simulink model "PROCESSOR"  (R2022b)
settings: Solver=FixedStepDiscrete  StartTime=0.0  StopTime=700  FixedStep=0.1  RelTol=1e-3  EnableMultiTasking=on
(part 2 of 2)

== stateflow chart PROCESSOR/Chart ==
  state SET_UP
    CODE_START=uint32(1);
    MEMORY=uint64(zeros([1 65536],"uint64"));
    MEMORY=STORE_INSTRUCTIONS(MEMORY,CODE_START);
    STACK_MIN=1025;
    STACK_MAX=8192;
    MEM_MIN=8193;
    MEM_MAX=64512;
    INTERUPT_TABLE=64513;
    RIP=CODE_START;
    RSP=uint32(8192);
    RBP=uint32(0);
    RCF=uint32(0);
    R=uint32(zeros([1 31],"uint32"));
    xR8=uint64(0);
    xR10=uint64(0);
    xR11=uint64(0);
    xR12=uint64(0);
    xR13=uint64(0);
    xR14=uint64(0);
    xR15=uint64(0);
  state FETCH
    state S128
      xR8=128;
    state S129
      xR8=129;
      sum=GET_REG(xR13,0,32);
    (default) -> S128
    S128 -> 1001 [order 1] : [~(GET_REG(RCF,3,5)==0)]
    S128 -> 999 [order 2] : [(GET_REG(RCF,3,5)==0)]{xR11=LOAD(MEMORY, RIP), xR13=SET_REG(xR13,0,32,uint64(RIP)),
        |  xR14=SET_REG(xR14,0,32,8), xR12=SET_REG(xR12,0,1,0), xR12=SET_REG(xR12,1,2,0),
        |  xR10=SET_REG(xR10,0,16,129)}
    1004 -> S129
    S129 -> 1057 : {RIP=uint32(sum)}
  state HALT
    state S0
      xR8=0;
    (default) -> S0
  state MULT
    state S69
      xR8=69;
      s=GET_REG(xR13,0,32);
      y_m=GET_REG(xR15,0,32);
      y_mNeg=GET_REG(xR12,6,7);
    state S68
      xR8=68;
      x_m=GET_REG(xR11,0,32);
      y_m=GET_REG(xR15,0,32);
      x_mNeg=GET_REG(xR12,5,6);
      y_mNeg=GET_REG(xR12,6,7);
    state S67
      xR8=67;
      x_m=GET_REG(xR11,0,32);
      y_m=GET_REG(xR15,0,32);
      x_m31=GET_REG(xR11,31,32);
      y_m31=GET_REG(xR15,31,32);
    state X
      svd=GET_REG(xR10,16,32);
    state S70
      xR8=70;
      s=GET_REG(xR13,0,32);
    state S1
      xR8=1;
      x_m=GET_REG(xR11,0,32);
      y_m0=GET_REG(xR15,0,1);
      y_m1=GET_REG(xR15,1,2);
    state S2
      xR8=2;
      s=GET_REG(xR13,0,32);
      co=GET_REG(xR12,2,3);
      x_m=GET_REG(xR11,0,32);
      y_mi=GET_REG(xR15,xR8,xR8+1);
    state ADDER
    state S3
      xR8=3;
      s=GET_REG(xR13,0,32);
      co=GET_REG(xR12,2,3);
      x_m=GET_REG(xR11,0,32);
      y_mi=GET_REG(xR15,xR8,xR8+1);
    state S4
      xR8=4;
      s=GET_REG(xR13,0,32);
      co=GET_REG(xR12,2,3);
      x_m=GET_REG(xR11,0,32);
      y_mi=GET_REG(xR15,xR8,xR8+1);
    state S5
      xR8=5;
      s=GET_REG(xR13,0,32);
      co=GET_REG(xR12,2,3);
      x_m=GET_REG(xR11,0,32);
      y_mi=GET_REG(xR15,xR8,xR8+1);
    state S6
      xR8=6;
      s=GET_REG(xR13,0,32);
      co=GET_REG(xR12,2,3);
      x_m=GET_REG(xR11,0,32);
      y_mi=GET_REG(xR15,xR8,xR8+1);
    state S7
      xR8=7;
      s=GET_REG(xR13,0,32);
      co=GET_REG(xR12,2,3);
      x_m=GET_REG(xR11,0,32);
      y_mi=GET_REG(xR15,xR8,xR8+1);
    state S8
      xR8=8;
      s=GET_REG(xR13,0,32);
      co=GET_REG(xR12,2,3);
      x_m=GET_REG(xR11,0,32);
      y_mi=GET_REG(xR15,xR8,xR8+1);
    state S9
      xR8=9;
      s=GET_REG(xR13,0,32);
      co=GET_REG(xR12,2,3);
      x_m=GET_REG(xR11,0,32);
      y_mi=GET_REG(xR15,xR8,xR8+1);
    state S10
      xR8=10;
      s=GET_REG(xR13,0,32);
      co=GET_REG(xR12,2,3);
      x_m=GET_REG(xR11,0,32);
      y_mi=GET_REG(xR15,xR8,xR8+1);
    state S11
      xR8=11;
      s=GET_REG(xR13,0,32);
      co=GET_REG(xR12,2,3);
      x_m=GET_REG(xR11,0,32);
      y_mi=GET_REG(xR15,xR8,xR8+1);
    state S12
      xR8=12;
      s=GET_REG(xR13,0,32);
      co=GET_REG(xR12,2,3);
      x_m=GET_REG(xR11,0,32);
      y_mi=GET_REG(xR15,xR8,xR8+1);
    state S13
      xR8=13;
      s=GET_REG(xR13,0,32);
      co=GET_REG(xR12,2,3);
      x_m=GET_REG(xR11,0,32);
      y_mi=GET_REG(xR15,xR8,xR8+1);
    state S14
      xR8=14;
      s=GET_REG(xR13,0,32);
      co=GET_REG(xR12,2,3);
      x_m=GET_REG(xR11,0,32);
      y_mi=GET_REG(xR15,xR8,xR8+1);
    state S15
      xR8=15;
      s=GET_REG(xR13,0,32);
      co=GET_REG(xR12,2,3);
      x_m=GET_REG(xR11,0,32);
      y_mi=GET_REG(xR15,xR8,xR8+1);
    state S16
      xR8=16;
      s=GET_REG(xR13,0,32);
      co=GET_REG(xR12,2,3);
      x_m=GET_REG(xR11,0,32);
      y_mi=GET_REG(xR15,xR8,xR8+1);
    state S17
      xR8=17;
      s=GET_REG(xR13,0,32);
      co=GET_REG(xR12,2,3);
      x_m=GET_REG(xR11,0,32);
      y_mi=GET_REG(xR15,xR8,xR8+1);
    state S18
      xR8=18;
      s=GET_REG(xR13,0,32);
      co=GET_REG(xR12,2,3);
      x_m=GET_REG(xR11,0,32);
      y_mi=GET_REG(xR15,xR8,xR8+1);
    state S19
      xR8=19;
      s=GET_REG(xR13,0,32);
      co=GET_REG(xR12,2,3);
      x_m=GET_REG(xR11,0,32);
      y_mi=GET_REG(xR15,xR8,xR8+1);
    state S20
      xR8=20;
      s=GET_REG(xR13,0,32);
      co=GET_REG(xR12,2,3);
      x_m=GET_REG(xR11,0,32);
      y_mi=GET_REG(xR15,xR8,xR8+1);
    state S21
      xR8=21;
      s=GET_REG(xR13,0,32);
      co=GET_REG(xR12,2,3);
      x_m=GET_REG(xR11,0,32);
      y_mi=GET_REG(xR15,xR8,xR8+1);
    state S22
      xR8=22;
      s=GET_REG(xR13,0,32);
      co=GET_REG(xR12,2,3);
      x_m=GET_REG(xR11,0,32);
      y_mi=GET_REG(xR15,xR8,xR8+1);
    state S23
      xR8=23;
      s=GET_REG(xR13,0,32);
      co=GET_REG(xR12,2,3);
      x_m=GET_REG(xR11,0,32);
      y_mi=GET_REG(xR15,xR8,xR8+1);
    state S24
      xR8=24;
      s=GET_REG(xR13,0,32);
      co=GET_REG(xR12,2,3);
      x_m=GET_REG(xR11,0,32);
      y_mi=GET_REG(xR15,xR8,xR8+1);
    state S25
      xR8=25;
      s=GET_REG(xR13,0,32);
      co=GET_REG(xR12,2,3);
      x_m=GET_REG(xR11,0,32);
      y_mi=GET_REG(xR15,xR8,xR8+1);
    state S26
      xR8=26;
      s=GET_REG(xR13,0,32);
      co=GET_REG(xR12,2,3);
      x_m=GET_REG(xR11,0,32);
      y_mi=GET_REG(xR15,xR8,xR8+1);
    state S27
      xR8=27;
      s=GET_REG(xR13,0,32);
      co=GET_REG(xR12,2,3);
      x_m=GET_REG(xR11,0,32);
      y_mi=GET_REG(xR15,xR8,xR8+1);
    state S28
      xR8=28;
      s=GET_REG(xR13,0,32);
      co=GET_REG(xR12,2,3);
      x_m=GET_REG(xR11,0,32);
      y_mi=GET_REG(xR15,xR8,xR8+1);
    state S29
      xR8=29;
      s=GET_REG(xR13,0,32);
      co=GET_REG(xR12,2,3);
      x_m=GET_REG(xR11,0,32);
      y_mi=GET_REG(xR15,xR8,xR8+1);
    state S30
      xR8=30;
      s=GET_REG(xR13,0,32);
      co=GET_REG(xR12,2,3);
      x_m=GET_REG(xR11,0,32);
      y_mi=GET_REG(xR15,xR8,xR8+1);
    state S31
      xR8=31;
      s=GET_REG(xR13,0,32);
      co=GET_REG(xR12,2,3);
      x_m=GET_REG(xR11,0,32);
      y_mi=GET_REG(xR15,xR8,xR8+1);
    state S71
      xR8=71;
      s=GET_REG(xR13,0,32);
      s31=GET_REG(xR13,31,32);
      co=GET_REG(xR12,2,3);
      x_mNeg=GET_REG(xR12,5,6);
      y_mNeg=GET_REG(xR12,6,7);
    state S73
      xR8=73;
      s=GET_REG(xR13,0,32);
      s31=GET_REG(xR13,31,32);
    state S72
      xR8=72;
    (junction 787) -> (junction 788)
    S67 -> (junction 787) [order 1] : [(y_m==1) & x_m & ~(x_m==1)]{
        | xR13=SET_REG(xR13,0,32,x_m),
        | xR12=SET_REG(xR12,7,8,x_m31),
        | xR12=SET_REG(xR12,8,9,0),
        | xR12=SET_REG(xR12,9,10,0)}
    (junction 788) -> (junction 790)
    (junction 802) -> (junction 804)
    (junction 795) -> (junction 802)
    (junction 800) -> (junction 795)
    S69 -> (junction 802) [order 1] : [y_mNeg]{
        | xR11=SET_REG(xR11,0,32,s),
        | xR13=SET_REG(xR13,0,32,0),
        | xR14=SET_REG(xR14,0,32,y_m),
        | xR12=SET_REG(xR12,1,2,0),
        | xR12=SET_REG(xR12,0,1,1),
        | xR10=SET_REG(xR10,0,16,70)}
    (junction 804) -> MULT.ADDER
    S68 -> (junction 795) [order 2] : [x_mNeg]{
        | xR13=SET_REG(xR13,0,32,0),
        | xR14=SET_REG(xR14,0,32,x_m),
        | xR12=SET_REG(xR12,1,2,0),
        | xR12=SET_REG(xR12,0,1,1),
        | xR10=SET_REG(xR10,0,16,69)}
    S68 -> (junction 800) [order 1] : [~x_mNeg & y_mNeg]{
        | xR13=SET_REG(xR13,0,32,0),
        | xR14=SET_REG(xR14,0,32,y_m),
        | xR12=SET_REG(xR12,1,2,0),
        | xR12=SET_REG(xR12,0,1,1),
        | xR10=SET_REG(xR10,0,16,70)}
    (junction 786) -> (junction 790)
    S67 -> (junction 786) [order 2] : [(x_m==1) & y_m & ~(y_m==1)]{
        | xR13=SET_REG(xR13,0,32,y_m),
        | xR12=SET_REG(xR12,7,8,y_m31),
        | xR12=SET_REG(xR12,8,9,0),
        | xR12=SET_REG(xR12,9,10,0)}
    (junction 790) -> MULT.X
    MULT.X -> 1377 [order 1] : [svd==195]
    MULT.X -> 1379 [order 2] : [svd==197]
    (default) -> S67
    447 -> S69
    S67 -> MULT.X [order 3] : [~x_m | ~y_m]{
        | xR13=SET_REG(xR13,0,32,0),
        | xR12=SET_REG(xR12,7,8,0),
        | xR12=SET_REG(xR12,8,9,0),
        | xR12=SET_REG(xR12,9,10,1)}
    S67 -> S68 [order 4] : [x_m & y_m & ~(x_m==1) & ~(y_m==1)]{
        | xR12=SET_REG(xR12,5,6,x_m31),
        | xR12=SET_REG(xR12,6,7,y_m31)}
    S73 -> MULT.X : {xR12=SET_REG(xR12,7,8,s31),
        | xR12=SET_REG(xR12,8,9,0)
        | xR12=SET_REG(xR12,9,10,~s)}
    S69 -> (junction 796) [order 2] : [~y_mNeg]{
        | xR11=SET_REG(xR11,0,32,s)}
    (junction 796) -> (junction 797)
    S68 -> S1 [order 3] : [~x_mNeg & ~y_mNeg]
    (junction 780) -> (junction 781)
    S1 -> (junction 780) [order 1] : [~y_m0 & ~y_m1]{
        | xR13=SET_REG(xR13,0,32,0)}
    (junction 781) -> (junction 779)
    (junction 778) -> (junction 779)
    S1 -> (junction 778) [order 2] : [~y_m0 & y_m1]{
        | xR13=SET_REG(xR13,0,32,bitsll(uint32(x_m),1))}
    (junction 779) -> S2
    453 -> S70
    463 -> S2
    (junction 797) -> S1
    S1 -> S2 [order 4] : [y_m0 & ~y_m1]{
        | xR13=SET_REG(xR13,0,32,x_m)}
    S70 -> S1 : {xR15=SET_REG(xR15,0,32,s)}
    S2 -> (junction 770) [order 3] : [(s | co)  & y_mi]{
        | xR14=SET_REG(xR14,0,32,bitsll(uint32(x_m),xR8)),
        | xR12=SET_REG(xR12,0,1,0),
        | xR12=SET_REG(xR12,1,2,co),
        | xR10=SET_REG(xR10,0,16,3)}
    (junction 770) -> (junction 771)
    S2 -> S3 [order 2] : [~s & ~co  & y_mi]{
        | xR13=SET_REG(xR13,0,32,bitsll(uint32(x_m),xR8))}
    S2 -> S3 [order 4] : [~s & ~co  & ~y_mi]{
        | xR13=SET_REG(xR13,0,32,0)}
    S1 -> (junction 768) [order 3] : [y_m0 & y_m1]{
        | xR13=SET_REG(xR13,0,32,x_m),
        | xR14=SET_REG(xR14,0,32,bitsll(uint32(x_m),1)),
        | xR12=SET_REG(xR12,0,1,0),
        | xR12=SET_REG(xR12,1,2,0),
        | xR10=SET_REG(xR10,0,16,2)}
    S2 -> (junction 772) [order 1] : [(s | co)  & ~y_mi]{
        | xR14=SET_REG(xR14,0,32,0),
        | xR12=SET_REG(xR12,0,1,0),
        | xR12=SET_REG(xR12,1,2,co),
        | xR10=SET_REG(xR10,0,16,3)}
    (junction 768) -> (junction 769)
    (junction 771) -> (junction 768)
    (junction 772) -> (junction 771)
    (junction 769) -> MULT.ADDER
    S3 -> MULT.ADDER [order 4] : [(s | co)  & y_mi]{
        | xR14=SET_REG(xR14,0,32,bitsll(uint32(x_m),xR8)),
        | xR12=SET_REG(xR12,0,1,0),
        | xR12=SET_REG(xR12,1,2,co),
        | xR10=SET_REG(xR10,0,16,4)}
    473 -> S3
    S3 -> MULT.ADDER [order 3] : [(s | co)  & ~y_mi]{
        | xR14=SET_REG(xR14,0,32,0),
        | xR12=SET_REG(xR12,0,1,0),
        | xR12=SET_REG(xR12,1,2,co),
        | xR10=SET_REG(xR10,0,16,4)}
    S3 -> S4 [order 2] : [~s & ~co  & y_mi]{
        | xR13=SET_REG(xR13,0,32,bitsll(uint32(x_m),xR8))}
    S3 -> S4 [order 1] : [~s & ~co  & ~y_mi]{
        | xR13=SET_REG(xR13,0,32,0)}
    MULT.ADDER -> 765
    S4 -> MULT.ADDER [order 4] : [(s | co)  & y_mi]{
        | xR14=SET_REG(xR14,0,32,bitsll(uint32(x_m),xR8)),
        | xR12=SET_REG(xR12,0,1,0),
        | xR12=SET_REG(xR12,1,2,co),
        | xR10=SET_REG(xR10,0,16,5)}
    483 -> S4
    S4 -> MULT.ADDER [order 3] : [(s | co)  & ~y_mi]{
        | xR14=SET_REG(xR14,0,32,0),
        | xR12=SET_REG(xR12,0,1,0),
        | xR12=SET_REG(xR12,1,2,co),
        | xR10=SET_REG(xR10,0,16,5)}
    S4 -> S5 [order 1] : [~s & ~co  & y_mi]{
        | xR13=SET_REG(xR13,0,32,bitsll(uint32(x_m),xR8))}
    S4 -> S5 [order 2] : [~s & ~co  & ~y_mi]{
        | xR13=SET_REG(xR13,0,32,0)}
    S5 -> MULT.ADDER [order 4] : [(s | co)  & y_mi]{
        | xR14=SET_REG(xR14,0,32,bitsll(uint32(x_m),xR8)),
        | xR12=SET_REG(xR12,0,1,0),
        | xR12=SET_REG(xR12,1,2,co),
        | xR10=SET_REG(xR10,0,16,6)}
    498 -> S5
    S5 -> MULT.ADDER [order 3] : [(s | co)  & ~y_mi]{
        | xR14=SET_REG(xR14,0,32,0),
        | xR12=SET_REG(xR12,0,1,0),
        | xR12=SET_REG(xR12,1,2,co),
        | xR10=SET_REG(xR10,0,16,6)}
    S5 -> S6 [order 2] : [~s & ~co  & y_mi]{
        | xR13=SET_REG(xR13,0,32,bitsll(uint32(x_m),xR8))}
    S5 -> S6 [order 1] : [~s & ~co  & ~y_mi]{
        | xR13=SET_REG(xR13,0,32,0)}
    S6 -> MULT.ADDER [order 4] : [(s | co)  & y_mi]{
        | xR14=SET_REG(xR14,0,32,bitsll(uint32(x_m),xR8)),
        | xR12=SET_REG(xR12,0,1,0),
        | xR12=SET_REG(xR12,1,2,co),
        | xR10=SET_REG(xR10,0,16,7)}
    496 -> S6
    S6 -> MULT.ADDER [order 3] : [(s | co)  & ~y_mi]{
        | xR14=SET_REG(xR14,0,32,0),
        | xR12=SET_REG(xR12,0,1,0),
        | xR12=SET_REG(xR12,1,2,co),
        | xR10=SET_REG(xR10,0,16,7)}
    S6 -> S7 [order 2] : [~s & ~co  & y_mi]{
        | xR13=SET_REG(xR13,0,32,bitsll(uint32(x_m),xR8))}
    S6 -> S7 [order 1] : [~s & ~co  & ~y_mi]{
        | xR13=SET_REG(xR13,0,32,0)}
    S7 -> MULT.ADDER [order 4] : [(s | co)  & y_mi]{
        | xR14=SET_REG(xR14,0,32,bitsll(uint32(x_m),xR8)),
        | xR12=SET_REG(xR12,0,1,0),
        | xR12=SET_REG(xR12,1,2,co),
        | xR10=SET_REG(xR10,0,16,8)}
    524 -> S7
    S7 -> MULT.ADDER [order 3] : [(s | co)  & ~y_mi]{
        | xR14=SET_REG(xR14,0,32,0),
        | xR12=SET_REG(xR12,0,1,0),
        | xR12=SET_REG(xR12,1,2,co),
        | xR10=SET_REG(xR10,0,16,8)}
    S7 -> S8 [order 2] : [~s & ~co  & y_mi]{
        | xR13=SET_REG(xR13,0,32,bitsll(uint32(x_m),xR8))}
    S7 -> S8 [order 1] : [~s & ~co  & ~y_mi]{
        | xR13=SET_REG(xR13,0,32,0)}
    S8 -> MULT.ADDER [order 4] : [(s | co)  & y_mi]{
        | xR14=SET_REG(xR14,0,32,bitsll(uint32(x_m),xR8)),
        | xR12=SET_REG(xR12,0,1,0),
        | xR12=SET_REG(xR12,1,2,co),
        | xR10=SET_REG(xR10,0,16,9)}
    S8 -> MULT.ADDER [order 3] : [(s | co)  & ~y_mi]{
        | xR14=SET_REG(xR14,0,32,0),
        | xR12=SET_REG(xR12,0,1,0),
        | xR12=SET_REG(xR12,1,2,co),
        | xR10=SET_REG(xR10,0,16,9)}
    522 -> S8
    S8 -> S9 [order 1] : [~s & ~co  & y_mi]{
        | xR13=SET_REG(xR13,0,32,bitsll(uint32(x_m),xR8))}
    S8 -> S9 [order 2] : [~s & ~co  & ~y_mi]{
        | xR13=SET_REG(xR13,0,32,0)}
    S9 -> MULT.ADDER [order 4] : [(s | co)  & y_mi]{
        | xR14=SET_REG(xR14,0,32,bitsll(uint32(x_m),xR8)),
        | xR12=SET_REG(xR12,0,1,0),
        | xR12=SET_REG(xR12,1,2,co),
        | xR10=SET_REG(xR10,0,16,10)}
    507 -> S9
    S9 -> MULT.ADDER [order 3] : [(s | co)  & ~y_mi]{
        | xR14=SET_REG(xR14,0,32,0),
        | xR12=SET_REG(xR12,0,1,0),
        | xR12=SET_REG(xR12,1,2,co),
        | xR10=SET_REG(xR10,0,16,10)}
    S9 -> S10 [order 2] : [~s & ~co  & y_mi]{
        | xR13=SET_REG(xR13,0,32,bitsll(uint32(x_m),xR8))}
    S9 -> S10 [order 1] : [~s & ~co  & ~y_mi]{
        | xR13=SET_REG(xR13,0,32,0)}
    S10 -> MULT.ADDER [order 4] : [(s | co)  & y_mi]{
        | xR14=SET_REG(xR14,0,32,bitsll(uint32(x_m),xR8)),
        | xR12=SET_REG(xR12,0,1,0),
        | xR12=SET_REG(xR12,1,2,co),
        | xR10=SET_REG(xR10,0,16,11)}
    503 -> S10
    S10 -> MULT.ADDER [order 3] : [(s | co)  & ~y_mi]{
        | xR14=SET_REG(xR14,0,32,0),
        | xR12=SET_REG(xR12,0,1,0),
        | xR12=SET_REG(xR12,1,2,co),
        | xR10=SET_REG(xR10,0,16,11)}
    S10 -> S11 [order 2] : [~s & ~co  & y_mi]{
        | xR13=SET_REG(xR13,0,32,bitsll(uint32(x_m),xR8))}
    S10 -> S11 [order 1] : [~s & ~co  & ~y_mi]{
        | xR13=SET_REG(xR13,0,32,0)}
    S11 -> MULT.ADDER [order 4] : [(s | co)  & y_mi]{
        | xR14=SET_REG(xR14,0,32,bitsll(uint32(x_m),xR8)),
        | xR12=SET_REG(xR12,0,1,0),
        | xR12=SET_REG(xR12,1,2,co),
        | xR10=SET_REG(xR10,0,16,12)}
    576 -> S11
    S11 -> MULT.ADDER [order 3] : [(s | co)  & ~y_mi]{
        | xR14=SET_REG(xR14,0,32,0),
        | xR12=SET_REG(xR12,0,1,0),
        | xR12=SET_REG(xR12,1,2,co),
        | xR10=SET_REG(xR10,0,16,12)}
    S11 -> S12 [order 2] : [~s & ~co  & y_mi]{
        | xR13=SET_REG(xR13,0,32,bitsll(uint32(x_m),xR8))}
    S11 -> S12 [order 1] : [~s & ~co  & ~y_mi]{
        | xR13=SET_REG(xR13,0,32,0)}
    S12 -> MULT.ADDER [order 3] : [(s | co)  & y_mi]{
        | xR14=SET_REG(xR14,0,32,bitsll(uint32(x_m),xR8)),
        | xR12=SET_REG(xR12,0,1,0),
        | xR12=SET_REG(xR12,1,2,co),
        | xR10=SET_REG(xR10,0,16,13)}
    574 -> S12
    S12 -> MULT.ADDER [order 2] : [(s | co)  & ~y_mi]{
        | xR14=SET_REG(xR14,0,32,0),
        | xR12=SET_REG(xR12,0,1,0),
        | xR12=SET_REG(xR12,1,2,co),
        | xR10=SET_REG(xR10,0,16,13)}
    S12 -> S13 [order 1] : [~s & ~co  & y_mi]{
        | xR13=SET_REG(xR13,0,32,bitsll(uint32(x_m),xR8))}
    S12 -> S13 [order 4] : [~s & ~co  & ~y_mi]{
        | xR13=SET_REG(xR13,0,32,0)}
    S13 -> MULT.ADDER [order 4] : [(s | co)  & y_mi]{
        | xR14=SET_REG(xR14,0,32,bitsll(uint32(x_m),xR8)),
        | xR12=SET_REG(xR12,0,1,0),
        | xR12=SET_REG(xR12,1,2,co),
        | xR10=SET_REG(xR10,0,16,14)}
    559 -> S13
    S13 -> MULT.ADDER [order 3] : [(s | co)  & ~y_mi]{
        | xR14=SET_REG(xR14,0,32,0),
        | xR12=SET_REG(xR12,0,1,0),
        | xR12=SET_REG(xR12,1,2,co),
        | xR10=SET_REG(xR10,0,16,14)}
    S13 -> S14 [order 2] : [~s & ~co  & y_mi]{
        | xR13=SET_REG(xR13,0,32,bitsll(uint32(x_m),xR8))}
    S13 -> S14 [order 1] : [~s & ~co  & ~y_mi]{
        | xR13=SET_REG(xR13,0,32,0)}
    S14 -> MULT.ADDER [order 4] : [(s | co)  & y_mi]{
        | xR14=SET_REG(xR14,0,32,bitsll(uint32(x_m),xR8)),
        | xR12=SET_REG(xR12,0,1,0),
        | xR12=SET_REG(xR12,1,2,co),
        | xR10=SET_REG(xR10,0,16,15)}
    S14 -> MULT.ADDER [order 3] : [(s | co)  & ~y_mi]{
        | xR14=SET_REG(xR14,0,32,0),
        | xR12=SET_REG(xR12,0,1,0),
        | xR12=SET_REG(xR12,1,2,co),
        | xR10=SET_REG(xR10,0,16,15)}
    555 -> S14
    S14 -> S15 [order 2] : [~s & ~co  & y_mi]{
        | xR13=SET_REG(xR13,0,32,bitsll(uint32(x_m),xR8))}
    S14 -> S15 [order 1] : [~s & ~co  & ~y_mi]{
        | xR13=SET_REG(xR13,0,32,0)}
    S15 -> MULT.ADDER [order 4] : [(s | co)  & y_mi]{
        | xR14=SET_REG(xR14,0,32,bitsll(uint32(x_m),xR8)),
        | xR12=SET_REG(xR12,0,1,0),
        | xR12=SET_REG(xR12,1,2,co),
        | xR10=SET_REG(xR10,0,16,16)}
    537 -> S15
    S15 -> MULT.ADDER [order 3] : [(s | co)  & ~y_mi]{
        | xR14=SET_REG(xR14,0,32,0),
        | xR12=SET_REG(xR12,0,1,0),
        | xR12=SET_REG(xR12,1,2,co),
        | xR10=SET_REG(xR10,0,16,16)}
    S15 -> S16 [order 2] : [~s & ~co  & y_mi]{
        | xR13=SET_REG(xR13,0,32,bitsll(uint32(x_m),xR8))}
    S15 -> S16 [order 1] : [~s & ~co  & ~y_mi]{
        | xR13=SET_REG(xR13,0,32,0)}
    S16 -> MULT.ADDER [order 3] : [(s | co)  & y_mi]{
        | xR14=SET_REG(xR14,0,32,bitsll(uint32(x_m),xR8)),
        | xR12=SET_REG(xR12,0,1,0),
        | xR12=SET_REG(xR12,1,2,co),
        | xR10=SET_REG(xR10,0,16,17)}
    542 -> S16
    S16 -> MULT.ADDER [order 4] : [(s | co)  & ~y_mi]{
        | xR14=SET_REG(xR14,0,32,0),
        | xR12=SET_REG(xR12,0,1,0),
        | xR12=SET_REG(xR12,1,2,co),
        | xR10=SET_REG(xR10,0,16,17)}
    S16 -> S17 [order 1] : [~s & ~co  & y_mi]{
        | xR13=SET_REG(xR13,0,32,bitsll(uint32(x_m),xR8))}
    S16 -> S17 [order 2] : [~s & ~co  & ~y_mi]{
        | xR13=SET_REG(xR13,0,32,0)}
    S17 -> MULT.ADDER [order 4] : [(s | co)  & y_mi]{
        | xR14=SET_REG(xR14,0,32,bitsll(uint32(x_m),xR8)),
        | xR12=SET_REG(xR12,0,1,0),
        | xR12=SET_REG(xR12,1,2,co),
        | xR10=SET_REG(xR10,0,16,18)}
    540 -> S17
    S17 -> MULT.ADDER [order 3] : [(s | co)  & ~y_mi]{
        | xR14=SET_REG(xR14,0,32,0),
        | xR12=SET_REG(xR12,0,1,0),
        | xR12=SET_REG(xR12,1,2,co),
        | xR10=SET_REG(xR10,0,16,18)}
    S17 -> S18 [order 2] : [~s & ~co  & y_mi]{
        | xR13=SET_REG(xR13,0,32,bitsll(uint32(x_m),xR8))}
    S17 -> S18 [order 1] : [~s & ~co  & ~y_mi]{
        | xR13=SET_REG(xR13,0,32,0)}
    S18 -> MULT.ADDER [order 3] : [(s | co)  & y_mi]{
        | xR14=SET_REG(xR14,0,32,bitsll(uint32(x_m),xR8)),
        | xR12=SET_REG(xR12,0,1,0),
        | xR12=SET_REG(xR12,1,2,co),
        | xR10=SET_REG(xR10,0,16,19)}
    S18 -> MULT.ADDER [order 4] : [(s | co)  & ~y_mi]{
        | xR14=SET_REG(xR14,0,32,0),
        | xR12=SET_REG(xR12,0,1,0),
        | xR12=SET_REG(xR12,1,2,co),
        | xR10=SET_REG(xR10,0,16,19)}
    551 -> S18
    S18 -> S19 [order 2] : [~s & ~co  & y_mi]{
        | xR13=SET_REG(xR13,0,32,bitsll(uint32(x_m),xR8))}
    S18 -> S19 [order 1] : [~s & ~co  & ~y_mi]{
        | xR13=SET_REG(xR13,0,32,0)}
    S19 -> MULT.ADDER [order 4] : [(s | co)  & y_mi]{
        | xR14=SET_REG(xR14,0,32,bitsll(uint32(x_m),xR8)),
        | xR12=SET_REG(xR12,0,1,0),
        | xR12=SET_REG(xR12,1,2,co),
        | xR10=SET_REG(xR10,0,16,20)}
    674 -> S19
    S19 -> MULT.ADDER [order 3] : [(s | co)  & ~y_mi]{
        | xR14=SET_REG(xR14,0,32,0),
        | xR12=SET_REG(xR12,0,1,0),
        | xR12=SET_REG(xR12,1,2,co),
        | xR10=SET_REG(xR10,0,16,20)}
    S19 -> S20 [order 2] : [~s & ~co  & y_mi]{
        | xR13=SET_REG(xR13,0,32,bitsll(uint32(x_m),xR8))}
    S19 -> S20 [order 1] : [~s & ~co  & ~y_mi]{
        | xR13=SET_REG(xR13,0,32,0)}
    S20 -> MULT.ADDER [order 4] : [(s | co)  & y_mi]{
        | xR14=SET_REG(xR14,0,32,bitsll(uint32(x_m),xR8)),
        | xR12=SET_REG(xR12,0,1,0),
        | xR12=SET_REG(xR12,1,2,co),
        | xR10=SET_REG(xR10,0,16,21)}
    S20 -> MULT.ADDER [order 3] : [(s | co)  & ~y_mi]{
        | xR14=SET_REG(xR14,0,32,0),
        | xR12=SET_REG(xR12,0,1,0),
        | xR12=SET_REG(xR12,1,2,co),
        | xR10=SET_REG(xR10,0,16,21)}
    672 -> S20
    S20 -> S21 [order 1] : [~s & ~co  & y_mi]{
        | xR13=SET_REG(xR13,0,32,bitsll(uint32(x_m),xR8))}
    S20 -> S21 [order 2] : [~s & ~co  & ~y_mi]{
        | xR13=SET_REG(xR13,0,32,0)}
    S21 -> MULT.ADDER [order 4] : [(s | co)  & y_mi]{
        | xR14=SET_REG(xR14,0,32,bitsll(uint32(x_m),xR8)),
        | xR12=SET_REG(xR12,0,1,0),
        | xR12=SET_REG(xR12,1,2,co),
        | xR10=SET_REG(xR10,0,16,22)}
    657 -> S21
    S21 -> MULT.ADDER [order 3] : [(s | co)  & ~y_mi]{
        | xR14=SET_REG(xR14,0,32,0),
        | xR12=SET_REG(xR12,0,1,0),
        | xR12=SET_REG(xR12,1,2,co),
        | xR10=SET_REG(xR10,0,16,22)}
    S21 -> S22 [order 2] : [~s & ~co  & y_mi]{
        | xR13=SET_REG(xR13,0,32,bitsll(uint32(x_m),xR8))}
    S21 -> S22 [order 1] : [~s & ~co  & ~y_mi]{
        | xR13=SET_REG(xR13,0,32,0)}
    S22 -> MULT.ADDER [order 3] : [(s | co)  & y_mi]{
        | xR14=SET_REG(xR14,0,32,bitsll(uint32(x_m),xR8)),
        | xR12=SET_REG(xR12,0,1,0),
        | xR12=SET_REG(xR12,1,2,co),
        | xR10=SET_REG(xR10,0,16,23)}
    S22 -> MULT.ADDER [order 4] : [(s | co)  & ~y_mi]{
        | xR14=SET_REG(xR14,0,32,0),
        | xR12=SET_REG(xR12,0,1,0),
        | xR12=SET_REG(xR12,1,2,co),
        | xR10=SET_REG(xR10,0,16,23)}
    607 -> S22
    S22 -> S23 [order 2] : [~s & ~co  & y_mi]{
        | xR13=SET_REG(xR13,0,32,bitsll(uint32(x_m),xR8))}
    S22 -> S23 [order 1] : [~s & ~co  & ~y_mi]{
        | xR13=SET_REG(xR13,0,32,0)}
    S23 -> MULT.ADDER [order 4] : [(s | co)  & y_mi]{
        | xR14=SET_REG(xR14,0,32,bitsll(uint32(x_m),xR8)),
        | xR12=SET_REG(xR12,0,1,0),
        | xR12=SET_REG(xR12,1,2,co),
        | xR10=SET_REG(xR10,0,16,24)}
    589 -> S23
    S23 -> MULT.ADDER [order 3] : [(s | co)  & ~y_mi]{
        | xR14=SET_REG(xR14,0,32,0),
        | xR12=SET_REG(xR12,0,1,0),
        | xR12=SET_REG(xR12,1,2,co),
        | xR10=SET_REG(xR10,0,16,24)}
    S23 -> S24 [order 2] : [~s & ~co  & y_mi]{
        | xR13=SET_REG(xR13,0,32,bitsll(uint32(x_m),xR8))}
    S23 -> S24 [order 1] : [~s & ~co  & ~y_mi]{
        | xR13=SET_REG(xR13,0,32,0)}
    S24 -> MULT.ADDER [order 4] : [(s | co)  & y_mi]{
        | xR14=SET_REG(xR14,0,32,bitsll(uint32(x_m),xR8)),
        | xR12=SET_REG(xR12,0,1,0),
        | xR12=SET_REG(xR12,1,2,co),
        | xR10=SET_REG(xR10,0,16,25)}
    S24 -> MULT.ADDER [order 3] : [(s | co)  & ~y_mi]{
        | xR14=SET_REG(xR14,0,32,0),
        | xR12=SET_REG(xR12,0,1,0),
        | xR12=SET_REG(xR12,1,2,co),
        | xR10=SET_REG(xR10,0,16,25)}
    594 -> S24
    S24 -> S25 [order 1] : [~s & ~co  & y_mi]{
        | xR13=SET_REG(xR13,0,32,bitsll(uint32(x_m),xR8))}
    S24 -> S25 [order 2] : [~s & ~co  & ~y_mi]{
        | xR13=SET_REG(xR13,0,32,0)}
    S25 -> MULT.ADDER [order 4] : [(s | co)  & y_mi]{
        | xR14=SET_REG(xR14,0,32,bitsll(uint32(x_m),xR8)),
        | xR12=SET_REG(xR12,0,1,0),
        | xR12=SET_REG(xR12,1,2,co),
        | xR10=SET_REG(xR10,0,16,26)}
    592 -> S25
    S25 -> MULT.ADDER [order 3] : [(s | co)  & ~y_mi]{
        | xR14=SET_REG(xR14,0,32,0),
        | xR12=SET_REG(xR12,0,1,0),
        | xR12=SET_REG(xR12,1,2,co),
        | xR10=SET_REG(xR10,0,16,26)}
    S25 -> S26 [order 2] : [~s & ~co  & y_mi]{
        | xR13=SET_REG(xR13,0,32,bitsll(uint32(x_m),xR8))}
    S25 -> S26 [order 1] : [~s & ~co  & ~y_mi]{
        | xR13=SET_REG(xR13,0,32,0)}
    S26 -> MULT.ADDER [order 4] : [(s | co)  & y_mi]{
        | xR14=SET_REG(xR14,0,32,bitsll(uint32(x_m),xR8)),
        | xR12=SET_REG(xR12,0,1,0),
        | xR12=SET_REG(xR12,1,2,co),
        | xR10=SET_REG(xR10,0,16,27)}
    S26 -> MULT.ADDER [order 3] : [(s | co)  & ~y_mi]{
        | xR14=SET_REG(xR14,0,32,0),
        | xR12=SET_REG(xR12,0,1,0),
        | xR12=SET_REG(xR12,1,2,co),
        | xR10=SET_REG(xR10,0,16,27)}
    603 -> S26
    S26 -> S27 [order 2] : [~s & ~co  & y_mi]{
        | xR13=SET_REG(xR13,0,32,bitsll(uint32(x_m),xR8))}
    S26 -> S27 [order 1] : [~s & ~co  & ~y_mi]{
        | xR13=SET_REG(xR13,0,32,0)}
    S27 -> MULT.ADDER [order 4] : [(s | co)  & y_mi]{
        | xR14=SET_REG(xR14,0,32,bitsll(uint32(x_m),xR8)),
        | xR12=SET_REG(xR12,0,1,0),
        | xR12=SET_REG(xR12,1,2,co),
        | xR10=SET_REG(xR10,0,16,28)}
    677 -> S27
    S27 -> MULT.ADDER [order 3] : [(s | co)  & ~y_mi]{
        | xR14=SET_REG(xR14,0,32,0),
        | xR12=SET_REG(xR12,0,1,0),
        | xR12=SET_REG(xR12,1,2,co),
        | xR10=SET_REG(xR10,0,16,28)}
    S27 -> S28 [order 2] : [~s & ~co  & y_mi]{
        | xR13=SET_REG(xR13,0,32,bitsll(uint32(x_m),xR8))}
    S27 -> S28 [order 1] : [~s & ~co  & ~y_mi]{
        | xR13=SET_REG(xR13,0,32,0)}
    S28 -> MULT.ADDER [order 4] : [(s | co)  & y_mi]{
        | xR14=SET_REG(xR14,0,32,bitsll(uint32(x_m),xR8)),
        | xR12=SET_REG(xR12,0,1,0),
        | xR12=SET_REG(xR12,1,2,co),
        | xR10=SET_REG(xR10,0,16,29)}
    S28 -> MULT.ADDER [order 3] : [(s | co)  & ~y_mi]{
        | xR14=SET_REG(xR14,0,32,0),
        | xR12=SET_REG(xR12,0,1,0),
        | xR12=SET_REG(xR12,1,2,co),
        | xR10=SET_REG(xR10,0,16,29)}
    676 -> S28
    S28 -> S29 [order 1] : [~s & ~co  & y_mi]{
        | xR13=SET_REG(xR13,0,32,bitsll(uint32(x_m),xR8))}
    S28 -> S29 [order 2] : [~s & ~co  & ~y_mi]{
        | xR13=SET_REG(xR13,0,32,0)}
    S29 -> MULT.ADDER [order 4] : [(s | co)  & y_mi]{
        | xR14=SET_REG(xR14,0,32,bitsll(uint32(x_m),xR8)),
        | xR12=SET_REG(xR12,0,1,0),
        | xR12=SET_REG(xR12,1,2,co),
        | xR10=SET_REG(xR10,0,16,30)}
    631 -> S29
    S29 -> MULT.ADDER [order 3] : [(s | co)  & ~y_mi]{
        | xR14=SET_REG(xR14,0,32,0),
        | xR12=SET_REG(xR12,0,1,0),
        | xR12=SET_REG(xR12,1,2,co),
        | xR10=SET_REG(xR10,0,16,30)}
    S29 -> S30 [order 2] : [~s & ~co  & y_mi]{
        | xR13=SET_REG(xR13,0,32,bitsll(uint32(x_m),xR8))}
    S29 -> S30 [order 1] : [~s & ~co  & ~y_mi]{
        | xR13=SET_REG(xR13,0,32,0)}
    S30 -> MULT.ADDER [order 1] : [(s | co)  & y_mi]{
        | xR14=SET_REG(xR14,0,32,bitsll(uint32(x_m),xR8)),
        | xR12=SET_REG(xR12,0,1,0),
        | xR12=SET_REG(xR12,1,2,co),
        | xR10=SET_REG(xR10,0,16,31)}
    S30 -> MULT.ADDER [order 2] : [(s | co)  & ~y_mi]{
        | xR14=SET_REG(xR14,0,32,0),
        | xR12=SET_REG(xR12,0,1,0),
        | xR12=SET_REG(xR12,1,2,co),
        | xR10=SET_REG(xR10,0,16,31)}
    629 -> S30
    S30 -> S31 [order 4] : [~s & ~co  & y_mi]{
        | xR13=SET_REG(xR13,0,32,bitsll(uint32(x_m),xR8))}
    S30 -> S31 [order 3] : [~s & ~co  & ~y_mi]{
        | xR13=SET_REG(xR13,0,32,0)}
    S31 -> MULT.ADDER [order 2] : [(s | co)  & y_mi]{
        | xR14=SET_REG(xR14,0,32,bitsll(uint32(x_m),xR8)),
        | xR12=SET_REG(xR12,0,1,0),
        | xR12=SET_REG(xR12,1,2,co),
        | xR10=SET_REG(xR10,0,16,71)}
    646 -> S31
    S31 -> MULT.ADDER [order 1] : [(s | co)  & ~y_mi]{
        | xR14=SET_REG(xR14,0,32,0),
        | xR12=SET_REG(xR12,0,1,0),
        | xR12=SET_REG(xR12,1,2,co),
        | xR10=SET_REG(xR10,0,16,71)}
    S31 -> S71 [order 3] : [~s & ~co  & y_mi]{
        | xR13=SET_REG(xR13,0,32,bitsll(uint32(x_m),xR8))}
    S31 -> S71 [order 4] : [~s & ~co  & ~y_mi]{
        | xR13=SET_REG(xR13,0,32,0)}
    822 -> S71
    S71 -> 827 [order 1] : [co | s31]{
        | RCF=uint32(SET_REG(RCF,3,5,1))}
    S71 -> S72 [order 3] : [~co & ~s31 & ((x_mNeg & ~y_mNeg) | (~x_mNeg & y_mNeg))]{
        | xR14=SET_REG(xR14,0,32,s)}
    S71 -> (junction 831) [order 2] : [~co & ~s31 & ((x_mNeg & y_mNeg) | (~x_mNeg & ~y_mNeg))]
    (junction 831) -> S73
    833 -> S73
    S72 -> MULT.ADDER : {xR13=SET_REG(xR13,0,32,0),
        | xR12=SET_REG(xR12,0,1,1),
        | xR12=SET_REG(xR12,1,2,0),
        | xR10=SET_REG(xR10,0,16,73)}
  state ADDER
    state S66
      xR8=66;
      x=GET_REG(xR13,0,32);
      y=GET_REG(xR14,0,32);
      x31=GET_REG(xR13,31,32);
      y31=GET_REG(xR14,31,32);
      ci=GET_REG(xR12,1,2);
    state S65
      xR8=65;
      ci=GET_REG(xR12,1,2);
      y=GET_REG(xR14,0,32);
      z=GET_REG(xR12,0,1);
    state S32
      xR8=32;
      i0=mod(xR8,uint64(32));
      i1=i0+1;
      co=GET_REG(xR12,2,3);
      ci=GET_REG(xR12,1,2);
      xi=GET_REG(xR13,i0,i1);
      yi=GET_REG(xR14,i0,i1);
    state S33
      xR8=33;
      i0=mod(xR8,uint64(32));
      i1=i0+1;
      co=GET_REG(xR12,2,3);
      ci=co;
      xi=GET_REG(xR13,i0,i1);
      yi=GET_REG(xR14,i0,i1);
    state S34
      xR8=34;
      i0=mod(xR8,uint64(32));
      i1=i0+1;
      co=GET_REG(xR12,2,3);
      ci=co;
      xi=GET_REG(xR13,i0,i1);
      yi=GET_REG(xR14,i0,i1);
    state S35
      xR8=35;
      i0=mod(xR8,uint64(32));
      i1=i0+1;
      co=GET_REG(xR12,2,3);
      ci=co;
      xi=GET_REG(xR13,i0,i1);
      yi=GET_REG(xR14,i0,i1);
    state S36
      xR8=36;
      i0=mod(xR8,uint64(32));
      i1=i0+1;
      co=GET_REG(xR12,2,3);
      ci=co;
      xi=GET_REG(xR13,i0,i1);
      yi=GET_REG(xR14,i0,i1);
    state S37
      xR8=37;
      i0=mod(xR8,uint64(32));
      i1=i0+1;
      co=GET_REG(xR12,2,3);
      ci=co;
      xi=GET_REG(xR13,i0,i1);
      yi=GET_REG(xR14,i0,i1);
    state S38
      xR8=38;
      i0=mod(xR8,uint64(32));
      i1=i0+1;
      co=GET_REG(xR12,2,3);
      ci=co;
      xi=GET_REG(xR13,i0,i1);
      yi=GET_REG(xR14,i0,i1);
    state S39
      xR8=39;
      i0=mod(xR8,uint64(32));
      i1=i0+1;
      co=GET_REG(xR12,2,3);
      ci=co;
      xi=GET_REG(xR13,i0,i1);
      yi=GET_REG(xR14,i0,i1);
    state S40
      xR8=40;
      i0=mod(xR8,uint64(32));
      i1=i0+1;
      co=GET_REG(xR12,2,3);
      ci=co;
      xi=GET_REG(xR13,i0,i1);
      yi=GET_REG(xR14,i0,i1);
    state S41
      xR8=41;
      i0=mod(xR8,uint64(32));
      i1=i0+1;
      co=GET_REG(xR12,2,3);
      ci=co;
      xi=GET_REG(xR13,i0,i1);
      yi=GET_REG(xR14,i0,i1);
    state S42
      xR8=42;
      i0=mod(xR8,uint64(32));
      i1=i0+1;
      co=GET_REG(xR12,2,3);
      ci=co;
      xi=GET_REG(xR13,i0,i1);
      yi=GET_REG(xR14,i0,i1);
    state S43
      xR8=43;
      i0=mod(xR8,uint64(32));
      i1=i0+1;
      co=GET_REG(xR12,2,3);
      ci=co;
      xi=GET_REG(xR13,i0,i1);
      yi=GET_REG(xR14,i0,i1);
    state S44
      xR8=44;
      i0=mod(xR8,uint64(32));
      i1=i0+1;
      co=GET_REG(xR12,2,3);
      ci=co;
      xi=GET_REG(xR13,i0,i1);
      yi=GET_REG(xR14,i0,i1);
    state S57
      xR8=57;
      i0=mod(xR8,uint64(32));
      i1=i0+1;
      co=GET_REG(xR12,2,3);
      ci=co;
      xi=GET_REG(xR13,i0,i1);
      yi=GET_REG(xR14,i0,i1);
    state S56
      xR8=56;
      i0=mod(xR8,uint64(32));
      i1=i0+1;
      co=GET_REG(xR12,2,3);
      ci=co;
      xi=GET_REG(xR13,i0,i1);
      yi=GET_REG(xR14,i0,i1);
    state S55
      xR8=55;
      i0=mod(xR8,uint64(32));
      i1=i0+1;
      co=GET_REG(xR12,2,3);
      ci=co;
      xi=GET_REG(xR13,i0,i1);
      yi=GET_REG(xR14,i0,i1);
    state S54
      xR8=54;
      i0=mod(xR8,uint64(32));
      i1=i0+1;
      co=GET_REG(xR12,2,3);
      ci=co;
      xi=GET_REG(xR13,i0,i1);
      yi=GET_REG(xR14,i0,i1);
    state S53
      xR8=53;
      i0=mod(xR8,uint64(32));
      i1=i0+1;
      co=GET_REG(xR12,2,3);
      ci=co;
      xi=GET_REG(xR13,i0,i1);
      yi=GET_REG(xR14,i0,i1);
    state S52
      xR8=52;
      i0=mod(xR8,uint64(32));
      i1=i0+1;
      co=GET_REG(xR12,2,3);
      ci=co;
      xi=GET_REG(xR13,i0,i1);
      yi=GET_REG(xR14,i0,i1);
    state S51
      xR8=51;
      i0=mod(xR8,uint64(32));
      i1=i0+1;
      co=GET_REG(xR12,2,3);
      ci=co;
      xi=GET_REG(xR13,i0,i1);
      yi=GET_REG(xR14,i0,i1);
    state S50
      xR8=50;
      i0=mod(xR8,uint64(32));
      i1=i0+1;
      co=GET_REG(xR12,2,3);
      ci=co;
      xi=GET_REG(xR13,i0,i1);
      yi=GET_REG(xR14,i0,i1);
    state S49
      xR8=49;
      i0=mod(xR8,uint64(32));
      i1=i0+1;
      co=GET_REG(xR12,2,3);
      ci=co;
      xi=GET_REG(xR13,i0,i1);
      yi=GET_REG(xR14,i0,i1);
    state S48
      xR8=48;
      i0=mod(xR8,uint64(32));
      i1=i0+1;
      co=GET_REG(xR12,2,3);
      ci=co;
      xi=GET_REG(xR13,i0,i1);
      yi=GET_REG(xR14,i0,i1);
    state S47
      xR8=47;
      i0=mod(xR8,uint64(32));
      i1=i0+1;
      co=GET_REG(xR12,2,3);
      ci=co;
      xi=GET_REG(xR13,i0,i1);
      yi=GET_REG(xR14,i0,i1);
    state S46
      xR8=46;
      i0=mod(xR8,uint64(32));
      i1=i0+1;
      co=GET_REG(xR12,2,3);
      ci=co;
      xi=GET_REG(xR13,i0,i1);
      yi=GET_REG(xR14,i0,i1);
    state S45
      xR8=45;
      i0=mod(xR8,uint64(32));
      i1=i0+1;
      co=GET_REG(xR12,2,3);
      ci=co;
      xi=GET_REG(xR13,i0,i1);
      yi=GET_REG(xR14,i0,i1);
    state S58
      xR8=58;
      i0=mod(xR8,uint64(32));
      i1=i0+1;
      co=GET_REG(xR12,2,3);
      ci=co;
      xi=GET_REG(xR13,i0,i1);
      yi=GET_REG(xR14,i0,i1);
    state S59
      xR8=59;
      i0=mod(xR8,uint64(32));
      i1=i0+1;
      co=GET_REG(xR12,2,3);
      ci=co;
      xi=GET_REG(xR13,i0,i1);
      yi=GET_REG(xR14,i0,i1);
    state S60
      xR8=60;
      i0=mod(xR8,uint64(32));
      i1=i0+1;
      co=GET_REG(xR12,2,3);
      ci=co;
      xi=GET_REG(xR13,i0,i1);
      yi=GET_REG(xR14,i0,i1);
    state S61
      xR8=61;
      i0=mod(xR8,uint64(32));
      i1=i0+1;
      co=GET_REG(xR12,2,3);
      ci=co;
      xi=GET_REG(xR13,i0,i1);
      yi=GET_REG(xR14,i0,i1);
    state S62
      xR8=62;
      i0=mod(xR8,uint64(32));
      i1=i0+1;
      co=GET_REG(xR12,2,3);
      ci=co;
      xi=GET_REG(xR13,i0,i1);
      yi=GET_REG(xR14,i0,i1);
    state S63i
      xR8=63;
      i0=mod(xR8,uint64(32));
      i1=i0+1;
      co=GET_REG(xR12,2,3);
      ci=co;
      xi=GET_REG(xR13,i0,i1);
      yi=GET_REG(xR14,i0,i1);
    state S63ii [commented out]
      xR8=63;
      x=GET_REG(xR13,0,32);
      x31=GET_REG(xR13,31,32);
      xNeg=GET_REG(xR12,3,4);
      yNeg=GET_REG(xR12,4,5);
    state S64
      xR8=64;
      x=GET_REG(xR13,0,32);
      x31=GET_REG(xR13,31,32);
      xNeg=GET_REG(xR12,3,4);
      yNeg=GET_REG(xR12,4,5);
    state X
      svd=GET_REG(xR10,0,16);
    (default) -> S65
    S65 -> S66 : {xR12=SET_REG(xR12,1,2,z | ci),
        | xR14=SET_REG(xR14,0,32, y * uint64(~z) + bitcmp(y) * z)  }
    S66 -> S32 [order 1] : [(x &  (y | ci)) | (y & (x | ci)) | (ci & (x | y))]{xR12=SET_REG(xR12,3,4,x31),
        | xR12=SET_REG(xR12,4,5,y31)}
    S41 -> S42 : {xR12=SET_REG(xR12,1,2,co),xR12=SET_REG(xR12,2,3,(xi & yi) | (ci & (xi | yi))),
        |  xR13=SET_REG(xR13,i0,i1,(~ci & ~xi & yi)  | (~ci & xi & ~yi) | (ci & ~xi & ~yi) | (ci & xi & yi))}
    S40 -> S41 : {xR12=SET_REG(xR12,1,2,co),xR12=SET_REG(xR12,2,3,(xi & yi) | (ci & (xi | yi))),
        |  xR13=SET_REG(xR13,i0,i1,(~ci & ~xi & yi)  | (~ci & xi & ~yi) | (ci & ~xi & ~yi) | (ci & xi & yi))}
    S38 -> S39 : {xR12=SET_REG(xR12,1,2,co),xR12=SET_REG(xR12,2,3,(xi & yi) | (ci & (xi | yi))),
        |  xR13=SET_REG(xR13,i0,i1,(~ci & ~xi & yi)  | (~ci & xi & ~yi) | (ci & ~xi & ~yi) | (ci & xi & yi))}
    S39 -> S40 : {xR12=SET_REG(xR12,1,2,co),xR12=SET_REG(xR12,2,3,(xi & yi) | (ci & (xi | yi))),
        |  xR13=SET_REG(xR13,i0,i1,(~ci & ~xi & yi)  | (~ci & xi & ~yi) | (ci & ~xi & ~yi) | (ci & xi & yi))}
    S34 -> S35 : {xR12=SET_REG(xR12,1,2,co),xR12=SET_REG(xR12,2,3,(xi & yi) | (ci & (xi | yi))),
        |  xR13=SET_REG(xR13,i0,i1,(~ci & ~xi & yi)  | (~ci & xi & ~yi) | (ci & ~xi & ~yi) | (ci & xi & yi))}
    S36 -> S37 : {xR12=SET_REG(xR12,1,2,co),xR12=SET_REG(xR12,2,3,(xi & yi) | (ci & (xi | yi))),
        |  xR13=SET_REG(xR13,i0,i1,(~ci & ~xi & yi)  | (~ci & xi & ~yi) | (ci & ~xi & ~yi) | (ci & xi & yi))}
    S37 -> S38 : {xR12=SET_REG(xR12,1,2,co),xR12=SET_REG(xR12,2,3,(xi & yi) | (ci & (xi | yi))),
        |  xR13=SET_REG(xR13,i0,i1,(~ci & ~xi & yi)  | (~ci & xi & ~yi) | (ci & ~xi & ~yi) | (ci & xi & yi))}
    S42 -> S43 : {xR12=SET_REG(xR12,1,2,co),xR12=SET_REG(xR12,2,3,(xi & yi) | (ci & (xi | yi))),
        |  xR13=SET_REG(xR13,i0,i1,(~ci & ~xi & yi)  | (~ci & xi & ~yi) | (ci & ~xi & ~yi) | (ci & xi & yi))}
    S43 -> S44 : {xR12=SET_REG(xR12,1,2,co),xR12=SET_REG(xR12,2,3,(xi & yi) | (ci & (xi | yi))),
        |  xR13=SET_REG(xR13,i0,i1,(~ci & ~xi & yi)  | (~ci & xi & ~yi) | (ci & ~xi & ~yi) | (ci & xi & yi))}
    S32 -> S33 : {xR12=SET_REG(xR12,2,3,(xi & yi) | (ci & (xi | yi))),
        | xR13=SET_REG(xR13,i0,i1,(~ci & ~xi & yi)  | (~ci & xi & ~yi) | (ci & ~xi & ~yi) | (ci & xi & yi))}
    S33 -> S34 : {xR12=SET_REG(xR12,1,2,co),xR12=SET_REG(xR12,2,3,(xi & yi) | (ci & (xi | yi))),
        |  xR13=SET_REG(xR13,i0,i1,(~ci & ~xi & yi)  | (~ci & xi & ~yi) | (ci & ~xi & ~yi) | (ci & xi & yi))}
    S35 -> S36 : {xR12=SET_REG(xR12,1,2,co),xR12=SET_REG(xR12,2,3,(xi & yi) | (ci & (xi | yi))),
        |  xR13=SET_REG(xR13,i0,i1,(~ci & ~xi & yi)  | (~ci & xi & ~yi) | (ci & ~xi & ~yi) | (ci & xi & yi))}
    S66 -> (junction 374) [order 3] : [~x & ~y]{
        | xR13=SET_REG(xR13,0,32,ci),
        | xR12=SET_REG(xR12,7,8,0),
        | xR12=SET_REG(xR12,8,9,0),
        | xR12=SET_REG(xR12,9,10,1)}
    S66 -> (junction 379) [order 4] : [~x & y & ~ci]{
        | xR13=SET_REG(xR13,0,32,y),
        | xR12=SET_REG(xR12,7,8,y31),
        | xR12=SET_REG(xR12,8,9,0),
        | xR12=SET_REG(xR12,9,10,0)}
    S44 -> S45 : {xR12=SET_REG(xR12,1,2,co),xR12=SET_REG(xR12,2,3,(xi & yi) | (ci & (xi | yi))),
        |  xR13=SET_REG(xR13,i0,i1,(~ci & ~xi & yi)  | (~ci & xi & ~yi) | (ci & ~xi & ~yi) | (ci & xi & yi))}
    (junction 374) -> (junction 376)
    (junction 379) -> (junction 381)
    S66 -> (junction 388) [order 2] : [x & ~y & ~ci]{
        | xR12=SET_REG(xR12,7,8,x31),
        | xR12=SET_REG(xR12,8,9,0),
        | xR12=SET_REG(xR12,9,10,0)}
    (junction 376) -> (junction 388)
    (junction 381) -> (junction 388)
    (junction 388) -> ADDER.X
    S56 -> S57 : {xR12=SET_REG(xR12,1,2,co),xR12=SET_REG(xR12,2,3,(xi & yi) | (ci & (xi | yi))),
        |  xR13=SET_REG(xR13,i0,i1,(~ci & ~xi & yi)  | (~ci & xi & ~yi) | (ci & ~xi & ~yi) | (ci & xi & yi))}
    S55 -> S56 : {xR12=SET_REG(xR12,1,2,co),xR12=SET_REG(xR12,2,3,(xi & yi) | (ci & (xi | yi))),
        |  xR13=SET_REG(xR13,i0,i1,(~ci & ~xi & yi)  | (~ci & xi & ~yi) | (ci & ~xi & ~yi) | (ci & xi & yi))}
    S54 -> S55 : {xR12=SET_REG(xR12,1,2,co),xR12=SET_REG(xR12,2,3,(xi & yi) | (ci & (xi | yi))),
        |  xR13=SET_REG(xR13,i0,i1,(~ci & ~xi & yi)  | (~ci & xi & ~yi) | (ci & ~xi & ~yi) | (ci & xi & yi))}
    S53 -> S54 : {xR12=SET_REG(xR12,1,2,co),xR12=SET_REG(xR12,2,3,(xi & yi) | (ci & (xi | yi))),
        |  xR13=SET_REG(xR13,i0,i1,(~ci & ~xi & yi)  | (~ci & xi & ~yi) | (ci & ~xi & ~yi) | (ci & xi & yi))}
    S57 -> S58 : {xR12=SET_REG(xR12,1,2,co),xR12=SET_REG(xR12,2,3,(xi & yi) | (ci & (xi | yi))),
        |  xR13=SET_REG(xR13,i0,i1,(~ci & ~xi & yi)  | (~ci & xi & ~yi) | (ci & ~xi & ~yi) | (ci & xi & yi))}
    S52 -> S53 : {xR12=SET_REG(xR12,1,2,co),xR12=SET_REG(xR12,2,3,(xi & yi) | (ci & (xi | yi))),
        |  xR13=SET_REG(xR13,i0,i1,(~ci & ~xi & yi)  | (~ci & xi & ~yi) | (ci & ~xi & ~yi) | (ci & xi & yi))}
    S51 -> S52 : {xR12=SET_REG(xR12,1,2,co),xR12=SET_REG(xR12,2,3,(xi & yi) | (ci & (xi | yi))),
        |  xR13=SET_REG(xR13,i0,i1,(~ci & ~xi & yi)  | (~ci & xi & ~yi) | (ci & ~xi & ~yi) | (ci & xi & yi))}
    S50 -> S51 : {xR12=SET_REG(xR12,1,2,co),xR12=SET_REG(xR12,2,3,(xi & yi) | (ci & (xi | yi))),
        |  xR13=SET_REG(xR13,i0,i1,(~ci & ~xi & yi)  | (~ci & xi & ~yi) | (ci & ~xi & ~yi) | (ci & xi & yi))}
    S49 -> S50 : {xR12=SET_REG(xR12,1,2,co),xR12=SET_REG(xR12,2,3,(xi & yi) | (ci & (xi | yi))),
        |  xR13=SET_REG(xR13,i0,i1,(~ci & ~xi & yi)  | (~ci & xi & ~yi) | (ci & ~xi & ~yi) | (ci & xi & yi))}
    S48 -> S49 : {xR12=SET_REG(xR12,1,2,co),xR12=SET_REG(xR12,2,3,(xi & yi) | (ci & (xi | yi))),
        |  xR13=SET_REG(xR13,i0,i1,(~ci & ~xi & yi)  | (~ci & xi & ~yi) | (ci & ~xi & ~yi) | (ci & xi & yi))}
    S47 -> S48 : {xR12=SET_REG(xR12,1,2,co),xR12=SET_REG(xR12,2,3,(xi & yi) | (ci & (xi | yi))),
        |  xR13=SET_REG(xR13,i0,i1,(~ci & ~xi & yi)  | (~ci & xi & ~yi) | (ci & ~xi & ~yi) | (ci & xi & yi))}
    S46 -> S47 : {xR12=SET_REG(xR12,1,2,co),xR12=SET_REG(xR12,2,3,(xi & yi) | (ci & (xi | yi))),
        |  xR13=SET_REG(xR13,i0,i1,(~ci & ~xi & yi)  | (~ci & xi & ~yi) | (ci & ~xi & ~yi) | (ci & xi & yi))}
    S45 -> S46 : {xR12=SET_REG(xR12,1,2,co),xR12=SET_REG(xR12,2,3,(xi & yi) | (ci & (xi | yi))),
        |  xR13=SET_REG(xR13,i0,i1,(~ci & ~xi & yi)  | (~ci & xi & ~yi) | (ci & ~xi & ~yi) | (ci & xi & yi))}
    (junction 1435) -> (junction 1437)
    (junction 1434) -> (junction 1435)
    (junction 1437) -> S64
    S60 -> S61 : {xR12=SET_REG(xR12,1,2,co),xR12=SET_REG(xR12,2,3,(xi & yi) | (ci & (xi | yi))),
        |  xR13=SET_REG(xR13,i0,i1,(~ci & ~xi & yi)  | (~ci & xi & ~yi) | (ci & ~xi & ~yi) | (ci & xi & yi))}
    S58 -> S59 : {xR12=SET_REG(xR12,1,2,co),xR12=SET_REG(xR12,2,3,(xi & yi) | (ci & (xi | yi))),
        |  xR13=SET_REG(xR13,i0,i1,(~ci & ~xi & yi)  | (~ci & xi & ~yi) | (ci & ~xi & ~yi) | (ci & xi & yi))}
    S61 -> S62 : {xR12=SET_REG(xR12,1,2,co),xR12=SET_REG(xR12,2,3,(xi & yi) | (ci & (xi | yi))),
        |  xR13=SET_REG(xR13,i0,i1,(~ci & ~xi & yi)  | (~ci & xi & ~yi) | (ci & ~xi & ~yi) | (ci & xi & yi))}
    S64 -> 344 [order 2] : [(x31 & ~xNeg & ~yNeg) | (~x31 & xNeg & yNeg)]{
        | RCF=uint32(SET_REG(RCF,3,5,1))}
    S59 -> S60 : {xR12=SET_REG(xR12,1,2,co),xR12=SET_REG(xR12,2,3,(xi & yi) | (ci & (xi | yi))),
        |  xR13=SET_REG(xR13,i0,i1,(~ci & ~xi & yi)  | (~ci & xi & ~yi) | (ci & ~xi & ~yi) | (ci & xi & yi))}
    S62 -> S63i : {xR12=SET_REG(xR12,1,2,co),xR12=SET_REG(xR12,2,3,(xi & yi) | (ci & (xi | yi))),
        |  xR13=SET_REG(xR13,i0,i1,(~ci & ~xi & yi)  | (~ci & xi & ~yi) | (ci & ~xi & ~yi) | (ci & xi & yi))}
    S63i -> (junction 1434) : {xR12=SET_REG(xR12,1,2,co),xR12=SET_REG(xR12,2,3,(xi & yi) | (ci & (xi | yi))),
        | xR13=SET_REG(xR13,i0,i1,(~ci & ~xi & yi)  | (~ci & xi & ~yi) | (ci & ~xi & ~yi) | (ci & xi & yi))}
    S63ii -> S64 [commented out] : {xR12=SET_REG(xR12,7,8,x31),
        | xR12=SET_REG(xR12,8,9,(x31 & ~xNeg & ~yNeg) | (~x31 & xNeg & yNeg))
        | xR12=SET_REG(xR12,9,10,~x)}
    S64 -> ADDER.X [order 1] : [~((x31 & ~xNeg & ~yNeg) | (~x31 & xNeg & yNeg))]
        | {xR12=SET_REG(xR12,7,8,x31),
        | xR12=SET_REG(xR12,9,10,~x)}
    ADDER.X -> 391 [order 1] : [svd==129]
    ADDER.X -> 857 [order 36] : [svd==2]
    ADDER.X -> 862 [order 31] : [svd==3]
    ADDER.X -> 861 [order 37] : [svd==4]
    ADDER.X -> 867 [order 33] : [svd==5]
    ADDER.X -> 871 [order 25] : [svd==6]
    ADDER.X -> 868 [order 16] : [svd==7]
    ADDER.X -> 876 [order 34] : [svd==8]
    ADDER.X -> 885 [order 27] : [svd==9]
    ADDER.X -> 878 [order 28] : [svd==10]
    ADDER.X -> 882 [order 26] : [svd==11]
    ADDER.X -> 886 [order 21] : [svd==12]
    ADDER.X -> 880 [order 7] : [svd==13]
    ADDER.X -> 894 [order 35] : [svd==14]
    ADDER.X -> 915 [order 30] : [svd==15]
    ADDER.X -> 908 [order 32] : [svd==16]
    ADDER.X -> 912 [order 29] : [svd==17]
    ADDER.X -> 916 [order 23] : [svd==18]
    ADDER.X -> 910 [order 13] : [svd==19]
    ADDER.X -> 896 [order 24] : [svd==20]
    ADDER.X -> 905 [order 19] : [svd==21]
    ADDER.X -> 898 [order 18] : [svd==22]
    ADDER.X -> 902 [order 15] : [svd==23]
    ADDER.X -> 906 [order 11] : [svd==24]
    ADDER.X -> 900 [order 5] : [svd==25]
    ADDER.X -> 944 [order 22] : [svd==26]
    ADDER.X -> 943 [order 20] : [svd==27]
    ADDER.X -> 929 [order 17] : [svd==28]
    ADDER.X -> 946 [order 9] : [svd==29]
    ADDER.X -> 935 [order 14] : [svd==30]
    ADDER.X -> 940 [order 12] : [svd==31]
    ADDER.X -> 936 [order 10] : [svd==69]
    ADDER.X -> 939 [order 8] : [svd==70]
    ADDER.X -> 938 [order 6] : [svd==71]
    ADDER.X -> 934 [order 4] : [svd==73]
    ADDER.X -> 1388 [order 3] : [svd==194]
    ADDER.X -> 1391 [order 2] : [svd==196]
  state DECODE
    state S161
      xR8=161;
    state S160
      xR8=160;
      icode=GET_REG(xR11,0,8);
      scal=GET_REG(xR11,23,27);
      ra=GET_REG(xR11,8,13);
      rb=GET_REG(xR11,13,18);
      rc=GET_REG(xR11,18,23);
      dest=GET_REG(xR11,8,40);
      disp18=GET_REG(xR11,18,50);
      disp27=GET_REG(xR11,27,59);
      imm=GET_REG(xR11,13,45);
      rest59=GET_REG(xR11,59,64);
      rest50=GET_REG(xR11,50,64);
      rest18=GET_REG(xR11,18,64);
      rest45=GET_REG(xR11,45,64);
      rest13=GET_REG(xR11,13,64);
      rest16=GET_REG(xR11,16,64);
      rest40=GET_REG(xR11,40,64);
      rest8=GET_REG(xR11,8,64);
    state S162
      xR8=162;
      reg_val=GET_REG(xR13,0,32);
    state S163
      xR8=163;
    state S164
      xR8=164;
      reg_val=GET_REG(xR13,0,32);
    state S165
      xR8=165;
    state S166
      xR8=166;
      reg_val=GET_REG(xR13,0,32);
    state S167
      xR8=167;
    state S168
      xR8=168;
      icode=GET_REG(xR11,0,8);
    (junction 1019) -> (junction 1021)
    S161 -> (junction 1019) [order 1] : [icode==77]{
        | RCF=uint32(SET_REG(RCF,3,5,0))}
    (junction 1021) -> 1013
    (default) -> S160
    S161 -> 1024 [order 2] : [icode==78]
    S160 -> 1013 [order 1] : [~(((icode>=0) & (icode<=2) & ((scal==1) | (scal==2) | (scal==4) | (scal==8)) & ~rest59) | ...
        | ((icode>=9) & (icode<=10) & ~rest50) | ...
        | ((icode>=17) & (icode<=33) & ~rest18) | ...
        | ((icode==44) & ~rest45) | ...
        | ((icode>=51) & (icode<=53) & ~rest13) | ...
        | ((icode==59) & ~rest16) | ...
        | ((icode>=60) & (icode<=67) & ~rest40) | ...
        | ((icode>=76) & (icode<=78) & ~rest8))]{RCF=uint32(SET_REG(RCF,3,5,2))}
    S160 -> S161 [order 2] : [((icode>=0) & (icode<=2) & ((scal==1) | (scal==2) | (scal==4) | (scal==8)) & ~rest59) | ...
        | ((icode>=9) & (icode<=10) & ~rest50) | ...
        | ((icode>=17) & (icode<=33) & ~rest18) | ...
        | ((icode==44) & ~rest45) | ...
        | ((icode>=51) & (icode<=53) & ~rest13) | ...
        | ((icode==59) & ~rest16) | ...
        | ((icode>=60) & (icode<=67) & ~rest40) | ...
        | ((icode>=76) & (icode<=78) & ~rest8)]{
        | xR12=SET_REG(xR12,15,23,icode),
        | xR12=SET_REG(xR12,23,28,ra),
        | xR12=SET_REG(xR12,28,32,scal),
        | xR12=SET_REG(xR12,32,64,dest)}
    S161 -> 1027 [order 3] : [(icode==1) | (icode==10) | ((icode>=24) & (icode<=33)) | (icode==51) | (icode==52)]{
        | xR13=SET_REG(xR13,0,1,0),
        | xR13=SET_REG(xR13,1,6,ra),
        | xR10=SET_REG(xR10,0,16,162)}
    (junction 1037) -> 1027
    S161 -> S163 [order 4] : [~((icode==1) | (icode==10) | ((icode>=24) & (icode<=33)) |  ...
        | (icode==51) | (icode==52) | (icode==77) | (icode==78))]
    1032 -> S162
    S162 -> S163 : {xR13=SET_REG(xR13,32,64,reg_val)}
    S163 -> (junction 1037) [order 1] : [((icode>=0) & (icode<=33))]{
        | xR13=SET_REG(xR13,0,1,0),
        | xR13=SET_REG(xR13,1,6,rb),
        | xR10=SET_REG(xR10,0,16,164)}
    (junction 1047) -> (junction 1037)
    S163 -> S165 [order 2] : [~((icode>=0) & (icode<=33))]
    1041 -> S164
    S164 -> S165 : {xR14=SET_REG(xR14,32,64,reg_val)}
    S165 -> (junction 1047) [order 1] : [((icode>=0) & (icode<=2))]{
        | xR13=SET_REG(xR13,0,1,0),
        | xR13=SET_REG(xR13,1,6,rc),
        | xR10=SET_REG(xR10,0,16,166)}
    S165 -> S167 [order 2] : [~((icode>=0) & (icode<=2))]
    1051 -> S166
    S167 -> S168 [order 1] : [(icode==9) | (icode==10)]{
        | xR12=SET_REG(xR12,32,64,disp18)}
    S168 -> 1068 [order 1] : [((icode>=0) & (icode<=2)) | (icode==9) | (icode==10) | ((icode>=24) & (icode<=33)) | ...
        |  ((icode>=51) & (icode<=53)) | (icode==59) | (icode==60) | (icode==76)]
    S166 -> S167 : {xR15=SET_REG(xR15,32,64,reg_val)}
    S167 -> S168 [order 2] : [(icode>=0) & (icode<=2)]{
        | xR12=SET_REG(xR12,32,64,disp27)}
    S167 -> S168 [order 3] : [(icode==44)]{
        | xR12=SET_REG(xR12,32,64,imm)}
    S168 -> 1074 [order 2] : [((icode>=17) & (icode<=23)) | (icode==44) | ((icode>=61) & (icode<=67))]
    S167 -> S168 [order 4] : [(icode==52) | (icode==53) | (icode==59) | (icode==60) | (icode==76)]{
        | xR14=SET_REG(xR14,32,64,RSP),
        | xR15=SET_REG(xR15,32,64,RIP)}
    S167 -> S168 [order 5] : [~((icode>=0) & (icode<=2)) & ~(icode==9) & ~(icode==10) & ~(icode==44) & ...
        | ~(icode==52) & ~(icode==53) & ~(icode==59) & ~(icode==60) & ~(icode==76)]
  state REG_FILE
    state S96
      xR8=96;
      wre=GET_REG(xR13,0,1);
      src=uint32(GET_REG(xR13,1,6));
      data_in=uint32(GET_REG(xR14,0,32));
    state S97
      xR8=97;
    state S98
      xR8=98;
    state X
      svd=GET_REG(xR10,0,16);
    (default) -> S96
    S96 -> S97 [order 1] : [~wre]
    S96 -> S98 [order 2] : [wre]
    S97 -> (junction 1117) : {xR13=SET_REG(xR13,0,32, ...
        |               (uint32((src >= 4) & (src <= 31)))*R(src) + uint32((src == 0))*RIP + ...
        |               uint32((src == 1))*RSP + uint32((src == 2))*RBP + uint32((src == 3))*RCF)}
    S98 -> (junction 1139) : {
        | RIP=uint32((src == 0))*data_in + uint32(~(src == 0))*RIP,
        | RSP=uint32((src == 1))*data_in + uint32(~(src == 1))*RSP,
        | RBP=uint32((src == 2))*data_in + uint32(~(src==2))*RBP,
        | RCF=uint32((src == 3))*data_in  + uint32(~(src == 3))*RCF,
        | R(src)=uint32(((src >= 4) & (src <= 31)))*data_in + uint32(~((src >= 4) & (src <= 31)))*R(src)
        | }
    (junction 1117) -> REG_FILE.X
    (junction 1139) -> REG_FILE.X
    REG_FILE.X -> 1143 [order 1] : [svd==162]
    REG_FILE.X -> 1144 [order 5] : [svd==164]
    REG_FILE.X -> 1145 [order 4] : [svd==166]
    REG_FILE.X -> 1364 [order 3] : [svd==257]
    REG_FILE.X -> 1367 [order 2] : [svd==258]
  state EXECUTION
    state ADDER
    state S192
      xR8=192;
      icode=GET_REG(xR12,15,23);
      val_a=uint32(GET_REG(xR13,32,64));
      val_b=uint32(GET_REG(xR14,32,64));
      val_c=uint32(GET_REG(xR12,32,64));
    state S193
      xR8=193;
      result=GET_REG(xR12,32,64);
      result31=GET_REG(xR12,63,64);
    state S195
      xR8=195;
      val_c=uint32(GET_REG(xR12,32,64));
    state S194
      xR8=194;
      icode=GET_REG(xR12,15,23);
      val_a=uint32(GET_REG(xR13,32,64));
      val_b=uint32(GET_REG(xR14,32,64));
      val_c=uint32(GET_REG(xR12,32,64));
      val_d=uint32(GET_REG(xR15,32,64));
      val_e=uint32(GET_REG(xR12,32,40));
      val_f=uint32(GET_REG(xR12,28,32));
      result=GET_REG(xR13,0,32);
    state MULT
    state S198
      xR8=198;
    state S196
      xR8=196;
      result=GET_REG(xR13,0,32);
    state S197
      xR8=197;
      result=GET_REG(xR13,0,32);
    EXECUTION.ADDER -> 1176
    (default) -> S192
    S192 -> S193 [order 1] : [icode==24]{xR12=SET_REG(xR12,32,64,bitand(val_a,val_b))}
    S193 -> (junction 1228) [order 1] : [result31]{
        | xR12=SET_REG(xR12,7,8,1),
        | xR12=SET_REG(xR12,8,9,0),
        | xR12=SET_REG(xR12,9,10,0)}
    S192 -> EXECUTION.ADDER [order 8] : [(icode==52) | (icode==59) | (icode==60)]{
        | xR13=SET_REG(xR13,0,32,val_b),
        | xR14=SET_REG(xR14,0,32,4),
        | xR12=SET_REG(xR12,0,1,1),
        | xR12=SET_REG(xR12,1,2,0)
        | xR10=SET_REG(xR10,0,16,194)}
    (junction 1228) -> (junction 1229)
    S192 -> S193 [order 2] : [icode==25]{xR12=SET_REG(xR12,32,64,bitor(val_a,val_b))}
    S192 -> S193 [order 3] : [icode==26]{xR12=SET_REG(xR12,32,64, bitor(bitand(val_a,bitcmp(val_b)), ...
        |                                                                      bitand(bitcmp(val_a),val_b)))}
    S193 -> (junction 1229) [order 2] : [~result]{
        | xR12=SET_REG(xR12,7,8,0),
        | xR12=SET_REG(xR12,8,9,0),
        | xR12=SET_REG(xR12,9,10,1)}
    S192 -> S193 [order 4] : [icode==27]{xR12=SET_REG(xR12,32,64,bitsll(val_a,mod(val_b,32)))}
    (junction 1229) -> (junction 1230)
    S192 -> EXECUTION.ADDER [order 9] : [(icode==53) | (icode==76)]{
        | xR13=SET_REG(xR13,0,32,val_b),
        | xR14=SET_REG(xR14,0,32,4),
        | xR12=SET_REG(xR12,0,1,0),
        | xR12=SET_REG(xR12,1,2,0)
        | xR10=SET_REG(xR10,0,16,194)}
    S192 -> S193 [order 5] : [icode==28]{xR12=SET_REG(xR12,32,64,bitsrl(val_a,mod(val_b,32)))}
    S192 -> S193 [order 6] : [icode==29]{xR12=SET_REG(xR12,32,64,sar(val_a,mod(val_b,32)))}
    S193 -> (junction 1230) [order 3] : [~result31 & result]{
        | xR12=SET_REG(xR12,7,8,0),
        | xR12=SET_REG(xR12,8,9,0),
        | xR12=SET_REG(xR12,9,10,0)}
    S192 -> S193 [order 7] : [icode==51]{xR12=SET_REG(xR12,32,64,bitcmp(val_a))}
    (junction 1230) -> (junction 1236)
    S192 -> EXECUTION.ADDER [order 10] : [((icode>=0) & (icode<=2)) | (icode==9) | (icode==10)]{
        | xR13=SET_REG(xR13,0,32,val_c),
        | xR14=SET_REG(xR14,0,32,val_b),
        | xR12=SET_REG(xR12,0,1,0),
        | xR12=SET_REG(xR12,1,2,0)
        | xR10=SET_REG(xR10,0,16,194)}
    S192 -> EXECUTION.ADDER [order 11] : [icode==30]{
        | xR13=SET_REG(xR13,0,32,val_a),
        | xR14=SET_REG(xR14,0,32,val_b),
        | xR12=SET_REG(xR12,0,1,0),
        | xR12=SET_REG(xR12,1,2,0)
        | xR10=SET_REG(xR10,0,16,194)}
    S192 -> (junction 1225) [order 13] : [icode==32]{
        | xR11=SET_REG(xR11,0,32,val_a),
        | xR15=SET_REG(xR15,0,32,val_b),
        | xR10=SET_REG(xR10,16,32,197)}
    (junction 1225) -> (junction 1189)
    S192 -> EXECUTION.ADDER [order 12] : [(icode==31) | (icode==33)]{
        | xR13=SET_REG(xR13,0,32,val_a),
        | xR14=SET_REG(xR14,0,32,val_b),
        | xR12=SET_REG(xR12,0,1,1),
        | xR12=SET_REG(xR12,1,2,0)
        | xR10=SET_REG(xR10,0,16,194)}
    (junction 1193) -> EXECUTION.ADDER
    S195 -> (junction 1193) [order 2] : [icode==59]{
        | xR14=SET_REG(xR14,0,32,INTERUPT_TABLE),
        | xR12=SET_REG(xR12,0,1,0),
        | xR12=SET_REG(xR12,1,2,0)
        | xR10=SET_REG(xR10,0,16,196)}
    (junction 1194) -> (junction 1193)
    1262 -> S195
    S195 -> (junction 1194) [order 1] : [(icode>=0) & (icode<=2)]{
        | xR14=SET_REG(xR14,0,32,val_c),
        | xR12=SET_REG(xR12,0,1,0),
        | xR12=SET_REG(xR12,1,2,0)
        | xR10=SET_REG(xR10,0,16,196)}
    EXECUTION.MULT -> 1186
    1253 -> S194
    S194 -> EXECUTION.MULT [order 1] : [icode==59]{
        | xR13=SET_REG(xR13,32,64,result),
        | xR11=SET_REG(xR11,0,32,val_e),
        | xR15=SET_REG(xR15,0,32,4),
        | xR10=SET_REG(xR10,16,32,195)}
    (junction 1189) -> EXECUTION.MULT
    S194 -> EXECUTION.MULT [order 2] : [(icode>=0) & (icode<=2)]{
        | xR12=SET_REG(xR12,32,64,result),
        | xR11=SET_REG(xR11,0,32,val_f),
        | xR15=SET_REG(xR15,0,32,val_d),
        | xR10=SET_REG(xR10,16,32,195)}
    S194 -> (junction 1203) [order 3] : [(icode==9) | (icode==10) | (icode==30) | (icode==31) | (icode==52) | (icode==53) | (icode==76)]{
        | xR12=SET_REG(xR12,32,64,result)}
    S194 -> (junction 1212) [order 5] : [icode==33]
    S194 -> (junction 1211) [order 4] : [icode==60]{
        | xR13=SET_REG(xR13,32,64,result)}
    (junction 1236) -> S198
    (junction 1203) -> (junction 1212)
    (junction 1212) -> (junction 1211)
    (junction 1211) -> S198
    1256 -> S196
    S196 -> S198 : {xR12=SET_REG(xR12,32,64,result)}
    S198 -> 1240 [order 1] : [(icode==0) | (icode==1) | (icode==9) | (icode==10) | (icode==52) | ...
        |  (icode==53) | (icode==59) | (icode==60) | (icode==76)]
    S198 -> 1242 [order 2] : [(icode==2) | (icode==51) | ((icode>=24) & (icode<=33))]
    1259 -> S197
    S197 -> S198 : {xR12=SET_REG(xR12,32,64,result)}
  state WRITE_BACK
    state REG_FILE
    state S256
      xR8=256;
      icode=GET_REG(xR12,15,23);
      ra=GET_REG(xR12,23,28);
      val_a=uint32(GET_REG(xR12,32,64));
      val_b=uint32(GET_REG(xR13,32,64));
      val_c=uint32(GET_REG(xR14,32,64));
      val_d=uint32(GET_REG(xR15,32,64));
      SF=GET_REG(RCF,0,1);
      ZF=GET_REG(RCF,2,3);
    state S257
      xR8=257;
      icode=GET_REG(xR12,15,23);
      ra=GET_REG(xR12,23,28);
      val_a=uint32(GET_REG(xR12,32,64));
      val_b=uint32(GET_REG(xR13,32,64));
      val_c=uint32(GET_REG(xR14,32,64));
      val_d=uint32(GET_REG(xR15,32,64));
      SF=GET_REG(RCF,0,1);
      ZF=GET_REG(RCF,2,3);
    state S258
      xR8=258;
      sf=GET_REG(xR12,7,8);
      zf=GET_REG(xR12,9,10);
    1352 -> S257
    (default) -> S256
    S256 -> S257 [order 6] : [(icode==52) | (icode==53) | (icode==76)]{
        | RSP=val_a}
    S256 -> WRITE_BACK.REG_FILE [order 5] : [(icode==0) | (icode==2) | (icode==9) | ((icode>=24) & (icode<=32)) | (icode==44) | (icode==51)]{
        | xR13=SET_REG(xR13,0,1,1),
        | xR13=SET_REG(xR13,1,6,ra),
        | xR14=SET_REG(xR14,0,32,val_a),
        | xR10=SET_REG(xR10,0,16,257)}
    S256 -> S257 [order 7] : [(icode==59) | (icode==60)]{
        | RSP=val_b}
    WRITE_BACK.REG_FILE -> 1314
    S256 -> WRITE_BACK.REG_FILE [order 1] : [(icode==17)]{
        | xR13=SET_REG(xR13,0,1,1),
        | xR13=SET_REG(xR13,1,6,ra),
        | xR14=SET_REG(xR14,0,32,val_c),
        | xR10=SET_REG(xR10,0,16,257)}
    S256 -> WRITE_BACK.REG_FILE [order 4] : [((icode==19) | (icode==21) | (icode==22)) & ZF]{
        | xR13=SET_REG(xR13,0,1,1),
        | xR13=SET_REG(xR13,1,6,ra),
        | xR14=SET_REG(xR14,0,32,val_c),
        | xR10=SET_REG(xR10,0,16,258)}
    S257 -> (junction 1344) [order 4] : [(icode==53)]{
        | xR13=SET_REG(xR13,0,1,1),
        | xR13=SET_REG(xR13,1,6,ra),
        | xR14=SET_REG(xR14,0,32,val_d),
        | xR10=SET_REG(xR10,0,16,258)}
    (junction 1344) -> (junction 1346)
    S256 -> S257 [order 11] : [((~(icode==20) & ~(icode==21) & ~(icode==23)) | SF  |  ZF) & ...
        | ((~(icode==18) & ~(icode==19) & ~(icode==23)) | ~SF) & ...
        | ((~(icode==19) & ~(icode==21) & ~(icode==22)) | ~ZF) & ...
        | ((~(icode==63) & ~(icode==65) & ~(icode==66)) | ~ZF) & ...
        | ((~(icode==62) & ~(icode==63) & ~(icode==67)) | ~SF) & ...
        | ((~(icode==64) & ~(icode==65) & ~(icode==67)) | SF | ZF) & ...
        | (~(icode==17)) & ...
        | (~(icode==0) & ~(icode==2) & ~(icode==9) & ~((icode>=24) & (icode<=32)) & ~(icode==44) & ~(icode==51)) & ...
        | (~(icode==52) & ~(icode==53) & ~(icode==76)) & ...
        | (~(icode==59) & ~(icode==60))]
    S256 -> WRITE_BACK.REG_FILE [order 3] : [((icode==18) | (icode==19) | (icode==23)) & SF]{
        | xR13=SET_REG(xR13,0,1,1),
        | xR13=SET_REG(xR13,1,6,ra),
        | xR14=SET_REG(xR14,0,32,val_c),
        | xR10=SET_REG(xR10,0,16,258)}
    S256 -> WRITE_BACK.REG_FILE [order 2] : [((icode==20) | (icode==21) | (icode==23)) & ~SF  &  ~ZF]{
        | xR13=SET_REG(xR13,0,1,1),
        | xR13=SET_REG(xR13,1,6,ra),
        | xR14=SET_REG(xR14,0,32,val_c),
        | xR10=SET_REG(xR10,0,16,258)}
    S256 -> S258 [order 10] : [((icode==63) | (icode==65) | (icode==66)) & ...
        | ZF]{
        | RIP=val_a}
    S256 -> S258 [order 9] : [((icode==62) | (icode==63) | (icode==67)) & ...
        | SF]{
        | RIP=val_a}
    S256 -> S258 [order 8] : [((icode==64) | (icode==65) | (icode==67)) & ...
        | ~SF & ~ZF]{
        | RIP=val_a}
    S257 -> (junction 1334) [order 1] : [(icode==59) | (icode==60) | (icode==61)]{
        | RIP=val_a}
    S257 -> (junction 1340) [order 3] : [(icode==76)]{
        | RIP=val_d}
    S257 -> (junction 1335) [order 2] : [~(icode==53) & ~(icode==59) & ~(icode==60) & ...
        |  ~(icode==61) & ~(icode==76)]
    1349 -> S258
    (junction 1334) -> S258
    (junction 1340) -> (junction 1334)
    (junction 1335) -> (junction 1340)
    S258 -> (junction 1357) [order 1] : [((icode>=24) & (icode<=33)) | (icode==51)]{
        | RCF=uint32(SET_REG(RCF,0,1,sf)),
        | RCF=uint32(SET_REG(RCF,2,3,zf)),
        | RCF=uint32(SET_REG(RCF,3,5,0))}
    (junction 1357) -> 1355
    (junction 1358) -> 1355
    S258 -> (junction 1358) [order 2] : [~((icode>=24) & (icode<=33)) & ~(icode==51)]{
        | RCF=uint32(SET_REG(RCF,0,1,0)),
        | RCF=uint32(SET_REG(RCF,2,3,0)),
        | RCF=uint32(SET_REG(RCF,3,5,0))}
    (junction 1346) -> WRITE_BACK.REG_FILE
  state MEMORY
    state S225
      xR8=225;
      val_a=uint32(GET_REG(xR12,32,64));
    state S224
      xR8=224;
      icode=GET_REG(xR12,15,23);
      val_a=uint32(GET_REG(xR12,32,64));
      val_b=uint32(GET_REG(xR13,32,64));
      val_c=uint32(GET_REG(xR14,32,64));
      val_d=uint32(GET_REG(xR15,32,64));
    state S226
      xR8=226;
    (default) -> S224
    S224 -> S225 [order 1] : [((icode==59) | (icode==60))& ...
        | ((val_c >=STACK_MIN) & (val_c<=STACK_MAX))]{
        | MEMORY=STORE(MEMORY,val_c,val_d)}
    S224 -> (junction 1281) [order 6] : [((icode==0) | (icode==1) | (icode==9) | (icode==10)) & ...
        | ~((val_a >=MEM_MIN) & (val_a<=MEM_MAX))]{
        | RCF=uint32(SET_REG(RCF,3,5,3))}
    (junction 1281) -> (junction 1282)
    S224 -> S225 [order 2] : [((icode==1) | (icode==10))& ...
        | ((val_a >=MEM_MIN) & (val_a<=MEM_MAX))]{
        | MEMORY=STORE(MEMORY,val_a,val_b)}
    S224 -> (junction 1282) [order 7] : [((icode==53) | (icode==76)) & ...
        | ~((val_a >=STACK_MIN) & (val_a<=STACK_MAX))]{
        | RCF=uint32(SET_REG(RCF,3,5,3))}
    (junction 1282) -> 1289
    (junction 1283) -> (junction 1282)
    S224 -> S225 [order 3] : [(icode==52)& ...
        | ((val_c >=STACK_MIN) & (val_c<=STACK_MAX))]{
        | MEMORY=STORE(MEMORY,val_c,val_b)}
    S224 -> (junction 1283) [order 8] : [((icode==52) | (icode==59) | (icode==60)) & ...
        | ~((val_c >=STACK_MIN) & (val_c<=STACK_MAX))]{
        | RCF=uint32(SET_REG(RCF,3,5,3))}
    S224 -> S225 [order 4] : [((icode==0) | (icode==9))& ...
        | ((val_a >=MEM_MIN) & (val_a<=MEM_MAX))]{
        | xR12=SET_REG(xR12,32,64,LOAD(MEMORY,val_a))}
    S224 -> S225 [order 5] : [((icode==53) | (icode==76))& ...
        | ((val_a >=STACK_MIN) & (val_a<=STACK_MAX))]{
        | xR15=SET_REG(xR15,32,64,LOAD(MEMORY,val_a))}
    S225 -> S226 [order 2] : [icode==59]{
        | xR12=SET_REG(xR12,32,64,LOAD(MEMORY,val_a))}
    S225 -> 1271 [order 1] : [~(icode==59)]
    S226 -> 1271
  (junction 1406) -> (junction 1408)
  (junction 1408) -> (junction 1407)
  1058 -> (junction 1406)
  (default) -> SET_UP
  (junction 1413) -> FETCH
  (junction 1417) -> (junction 1413)
  1025 -> (junction 1413)
  (junction 1416) -> (junction 1417)
  SET_UP -> FETCH
  1002 -> HALT
  (junction 1422) -> HALT
  (junction 1421) -> (junction 1422)
  1000 -> ADDER
  392 -> 1005
  462 -> HALT
  766 -> ADDER
  345 -> HALT
  859 -> 464
  864 -> 474
  865 -> 485
  872 -> 682
  1014 -> HALT
  873 -> 731
  874 -> 732
  887 -> 733
  888 -> 734
  889 -> 735
  890 -> 736
  891 -> 737
  892 -> 738
  917 -> 739
  918 -> 740
  919 -> 741
  (junction 1407) -> DECODE
  920 -> 742
  921 -> 743
  922 -> 744
  1028 -> REG_FILE
  923 -> 745
  924 -> 746
  1149 -> 1033
  925 -> 747
  926 -> 748
  1150 -> 1043
  927 -> 749
  1151 -> 1052
  928 -> 750
  949 -> 751
  950 -> 752
  951 -> 753
  952 -> 754
  953 -> 755
  954 -> 756
  1315 -> REG_FILE
  955 -> 448
  1366 -> 1353
  1369 -> 1350
  956 -> 455
  957 -> 823
  1069 -> (junction 1403)
  1075 -> (junction 1396)
  958 -> 834
  (junction 1383) -> MULT
  (junction 1372) -> (junction 1383)
  1177 -> ADDER
  1390 -> 1254
  1393 -> 1257
  1380 -> 1263
  1378 -> 1260
  (junction 1403) -> EXECUTION
  1356 -> (junction 1416)
  1243 -> (junction 1396)
  (junction 1396) -> WRITE_BACK
  1272 -> (junction 1396)
  1187 -> (junction 1372)
  1241 -> MEMORY
  1290 -> (junction 1421)
  data: INSTRUCTION function_output; ICODE function_input; RA function_input; RB function_input; RC function_input; S function_input; D function_input; MEM function_input; DATA function_output; ADDR function_input; IN_xREG function_input; START_BIT function_input; END_BIT function_input; OUT_xREG function_output; VALUE function_input; OUT function_output; MEM function_input; M_START function_input; IN_xREG function_input; START_BIT function_input; END_BIT function_input; VALUE function_output; MEM function_input; ADDR function_input; DATA function_input; OUT function_output; val_1 function_input; val_2 function_input; out function_output; src function_input; RIP_IN function_input; data_out function_output; RSP_IN function_input; RBP_IN function_input; RCF_IN function_input; R_IN function_input; MEMORY local uint64 size=[1 65536]; xR8 local uint64; RIP local uint32; xR10 local uint64; xR12 local uint64; xR13 local uint64; xR14 local uint64; RCF local uint32; xR11 local uint64; ci local; i0 local; co local; i1 local; of local; x local; x31 local; xNeg local; xi local; y local; y31 local; yNeg local; yi local; z local; s local; x_m local; xR15 local; x_m31 local; x_mNeg local; y_m local; y_m0 local; y_m1 local; y_m31 local; y_mNeg local; y_mi local; s31 local; svd local; dest local; disp18 local; disp27 local; icode local; imm local; ra local; rb local; rc local; reg_val local; rest13 local; rest16 local; rest18 local; rest40 local; rest45 local; rest50 local; rest59 local; rest8 local; scal local; sum local; RSP local; wre local; data_in local; RBP local; R local; src local; val_a local; val_b local; result local; result31 local; val_c local; val_d local; val_e local; val_f local; INTERUPT_TABLE local; MEM_MAX local; MEM_MIN local; STACK_MAX local; STACK_MIN local; SF local; ZF local; sf local; zf local; CODE_START local
  function INSTRUCTION = MAKE_INSTRUCT(ICODE,RA,RB,RC,S,D):
    | function INSTRUCTION = MAKE_INSTRUCT(ICODE,RA,RB,RC,S,D)
    |     
    |     INSTRUCTION=uint64(0);
    |     shft_val=0;
    | 
    |     if (ICODE~=0xFFFFFFFFFFFFFFFF)
    |         INSTRUCTION=bitor(INSTRUCTION,bitsll(ICODE,shft_val),"uint64");
    |         shft_val=shft_val+8;
    |     end
    |     if (RA~=0xFFFFFFFFFFFFFFFF)
    |         INSTRUCTION=bitor(INSTRUCTION,bitsll(RA,shft_val),"uint64");
    |         shft_val=shft_val+5;
    |     end
    |     if (RB~=0xFFFFFFFFFFFFFFFF)
    |         INSTRUCTION=bitor(INSTRUCTION,bitsll(RB,shft_val),"uint64");
    |         shft_val=shft_val+5;
    |     end
    |     if (RC~=0xFFFFFFFFFFFFFFFF)
    |         INSTRUCTION=bitor(INSTRUCTION,bitsll(RC,shft_val),"uint64");
    |         shft_val=shft_val+5;
    |     end
    |     if (S~=0xFFFFFFFFFFFFFFFF)
    |         INSTRUCTION=bitor(INSTRUCTION,bitsll(S,shft_val),"uint64");
    |         shft_val=shft_val+4;
    |     end
    |     if (D~=0xFFFFFFFFFFFFFFFF)
    |         INSTRUCTION=bitor(INSTRUCTION,bitsll(uint64(D),shft_val),"uint64");
    |         %shft_val=shft_val+32;
    |     end
    |     
    | end
  function DATA = LOAD(MEM,ADDR):
    | function DATA = LOAD(MEM,ADDR)
    | 
    |     DATA=MEM(ADDR);
    |     
    | end
  function OUT_xREG = SET_REG(IN_xREG,START_BIT,END_BIT,VALUE):
    | function OUT_xREG = SET_REG(IN_xREG,START_BIT,END_BIT,VALUE)
    |     %bitor(bitand(xR10,0xFFFFFFFFFFFF0000,"uint64"),uint64(129),"uint64")
    |     
    |     IS_64=uint64(END_BIT==64);
    |     
    |     END_BIT=mod(uint64(END_BIT),uint64(64));
    | 
    |     chunk_start=bitsll(uint64(0xFFFFFFFFFFFFFFFF),uint64(START_BIT));
    | 
    | 
    |     chunk_end=bitsll(uint64(0xFFFFFFFFFFFFFFFF),uint64(END_BIT));
    |     chunk_end=bitcmp(uint64(chunk_end));
    | 
    |     chunk_end=IS_64*uint64(0xFFFFFFFFFFFFFFFF) + uint64(~IS_64)*chunk_end;
    |     
    |     chunk=bitand(uint64(chunk_start),uint64(chunk_end),"uint64");
    |     
    |     VALUE=bitand(uint64(VALUE),uint64(bitsrl(chunk,START_BIT)));
    |     VALUE=bitsll(uint64(VALUE),uint64(START_BIT));
    |     
    | 
    |     chunk=bitcmp(uint64(chunk));  
    | 
    | 
    |     IN_xREG=bitand(uint64(IN_xREG),uint64(chunk),"uint64");
    | 
    | 
    | 
    |     OUT_xREG=bitor(uint64(IN_xREG),uint64(VALUE),"uint64");
    | 
    | end
  function OUT = STORE_INSTRUCTIONS(MEM,M_START):
    | function OUT = STORE_INSTRUCTIONS(MEM,M_START)
    |     %coder.extrinsic('containers.Map')
    |     %global i;
    |     %global MEM_START;
    |     %global MEMORY;
    |     %i=uint64(0);
    |     
    |     NUM_OF_INSTRUCTIONS = 14;
    |     SP=0xFFFFFFFFFFFFFFFF;
    |     
    |     %FUNCTION MULT
    | 
    |     %PUSH RBP
    |     MEM(8193) = MAKE_INSTRUCT(52,2,SP,SP,SP,SP);
    |     %MOV RBP, RSP
    |     MEM(8193+8) = MAKE_INSTRUCT(17,2,1,SP,SP,SP);
    |     %MULT R5, R6
    |     MEM(8193+16) = MAKE_INSTRUCT(32,5,6,SP,SP,SP);
    |     %MOV R4, R5
    |     MEM(8193+24) = MAKE_INSTRUCT(17,4,5,SP,SP,SP);
    |     %MOV RSP, RBP
    |     MEM(8193+32) = MAKE_INSTRUCT(17,1,2,SP,SP,SP);
    |     %POP RBP
    |     MEM(8193+40) = MAKE_INSTRUCT(53,2,SP,SP,SP,SP);
    |     %RET
    |     MEM(8193+48) = MAKE_INSTRUCT(76,SP,SP,SP,SP,SP);
    | 
    |     %FUNCTION ADD
    | 
    |     %PUSH RBP
    |     MEM(8193+64) = MAKE_INSTRUCT(52,2,SP,SP,SP,SP);
    |     %MOV RBP, RSP
    |     MEM(8193+72) = MAKE_INSTRUCT(17,2,1,SP,SP,SP);
    |     %ADD R5, R6
    |     MEM(8193+80) = MAKE_INSTRUCT(30,5,6,SP,SP,SP);
    |     %MOV R4, R5
    |     MEM(8193+88) = MAKE_INSTRUCT(17,4,5,SP,SP,SP);
    |     %MOV RSP, RBP
    |     MEM(8193+96) = MAKE_INSTRUCT(17,1,2,SP,SP,SP);
    |     %POP RBP
    |     MEM(8193+104) = MAKE_INSTRUCT(53,2,SP,SP,SP,SP);
    |     %RET
    |     MEM(8193+112) = MAKE_INSTRUCT(76,SP,SP,SP,SP,SP);
    | 
    | 
    |     INSTRUCTIONS = zeros([1 128]);
    |     %MOV R5, 7
    |     INSTRUCTIONS(1)=MAKE_INSTRUCT(44,5,SP,SP,SP,7);
    |     %MOV R7, 13
    |     INSTRUCTIONS(2)=MAKE_INSTRUCT(44,7,SP,SP,SP,13);
    |     %MOV R8, 56
    |     INSTRUCTIONS(3)=MAKE_INSTRUCT(44,8,SP,SP,SP,56);
    |     %MOV MEM(8193+56),R7
    |     INSTRUCTIONS(4)=MAKE_INSTRUCT(10,7,8,SP,SP,8193);
    |     %MOV R7,8
    |     INSTRUCTIONS(5)=MAKE_INSTRUCT(44,7,SP,SP,SP,8);
    |     %MOV R8,6
    |     INSTRUCTIONS(6)=MAKE_INSTRUCT(44,8,SP,SP,SP,6);
    |     %MOV R6,MEM(8193+56)
    |     INSTRUCTIONS(7)=MAKE_INSTRUCT(0,6,7,8,8,8193);
    |     %MOV R10, 74
    |     INSTRUCTIONS(8)=MAKE_INSTRUCT(44,10,SP,SP,SP,74);
    |     %MOV R11, 72
    |     INSTRUCTIONS(9)=MAKE_INSTRUCT(44,11,SP,SP,SP,72);
    |     %CMP R10, R11
    |     INSTRUCTIONS(10)=MAKE_INSTRUCT(33,10,11,SP,SP,SP);
    |     %JMPG (TO CALL ADD)
    |     INSTRUCTIONS(11)=MAKE_INSTRUCT(64,SP,SP,SP,SP,97);
    |     %CALL 8193 (MULT)
    |     INSTRUCTIONS(12)=MAKE_INSTRUCT(60,SP,SP,SP,SP,8193);
    |     %CALL 8257 (ADD)
    |     INSTRUCTIONS(13)=MAKE_INSTRUCT(60,SP,SP,SP,SP,8257);
    |     %HALT
    |     INSTRUCTIONS(14)=MAKE_INSTRUCT(77,SP,SP,SP,SP,SP);
    | 
    |     
    |     %MEM_START = uint32(1);
    | 
    |     for i= uint32(0):NUM_OF_INSTRUCTIONS
    |     
    |         MEM(M_START+uint32(8)*i)=INSTRUCTIONS(uint32(1)+i);
    |     end
    | 
    |     OUT=MEM;
    | end
  function VALUE = GET_REG(IN_xREG,START_BIT,END_BIT):
    | function VALUE = GET_REG(IN_xREG,START_BIT,END_BIT)
    |     
    |     IS_64=uint64(END_BIT==64);
    |     
    |     END_BIT=mod(uint64(END_BIT),uint64(64));
    | 
    |     chunk_start=bitsll(uint64(0xFFFFFFFFFFFFFFFF),uint64(START_BIT));
    | 
    |     chunk_end=bitcmp(bitsll(uint64(0xFFFFFFFFFFFFFFFF),uint64(END_BIT)));
    |     
    |     chunk_end=IS_64*uint64(0xFFFFFFFFFFFFFFFF) + uint64(~IS_64)*chunk_end;
    | 
    |     chunk=bitand(uint64(chunk_start),uint64(chunk_end),"uint64");
    | 
    |     IN_xREG=bitand(uint64(IN_xREG),uint64(chunk),"uint64");
    | 
    |     VALUE=bitsrl(uint64(IN_xREG),START_BIT);
    | 
    | end
  function OUT = STORE(MEM,ADDR,DATA):
    | function OUT = STORE(MEM,ADDR,DATA)
    | 
    |     MEM(ADDR)=uint64(DATA);
    |     
    |     OUT=MEM;
    | end
  function out = sar(val_1,val_2):
    | function out = sar(val_1,val_2)
    | 
    |     n=mod(uint32(val_2),32);
    | 
    |     out=bitsrl(uint32(val_1),n);
    | 
    |     carry=bitsrl(uint32(0xFFFFFFFF),n);
    | 
    |     carry=bitcmp(uint32(carry));
    | 
    |     carry=uint32(GET_REG(val_1,31,32))*carry;
    | 
    |     out=bitor(uint32(out),carry);
    | 
    | 
    | end
  function data_out = read_reg(src,RIP_IN,RSP_IN,RBP_IN,RCF_IN,R_IN):
    | function data_out = read_reg(src,RIP_IN,RSP_IN,RBP_IN,RCF_IN,R_IN)
    |     
    |    data_out= ((src >= 4) & (src <= 31))*R_IN(src) + (src == 0)*RIP_IN + ...
    |               (src == 1)*RSP_IN + (src == 2)*RBP_IN + (src == 3)*RCF_IN;
    |     
    |   %{ 
    |    if ((src >= 4) && (src <= 31)) 
    |         data_out=R_IN(src);
    |     elseif (src == 0)
    |         data_out=RIP_IN;
    |     elseif (src == 1)
    |         data_out=RSP_IN;
    |     elseif (src == 2)
    |         data_out=RBP_IN;
    |     elseif (src == 3)
    |         data_out=RCF_IN;
    |     end
    |   %}
    | 
    | end
